simulink model "GridN1"  (R2021a)
settings: Solver=FixedStepAuto  StartTime=0  StopTime=0.2  FixedStep=0.2  RelTol=1e-3
libraries: spsDistributedParametersLineLib x45, spsThreePhaseSeriesRLCLoadLib x20, spsThreePhaseVIMeasurementLib x3, spsGroundLib x1, spsThreePhaseSourceLib x1, spsSeriesRLCBranchLib x1, spspowerguiLib x1
settings Model: Creator=miair  LastModifiedBy=Admin
settings SolverCC: AlgebraicLoopSolver=TrustRegion
settings DebuggingCC: SFMachineParentedDataDiag=warning  ArithmeticOperatorsInVariantConditions=warning
settings SFSimCC: SimUseLocalCustomCode=off  CustomCodeUndefinedFunction=UseInterfaceOnly
settings RTWCC: RTWUseLocalCustomCode=off
settings CodeAppCC: StateflowObjectComments=on
settings SimscapeCC: SimscapeNormalizeSystem=off

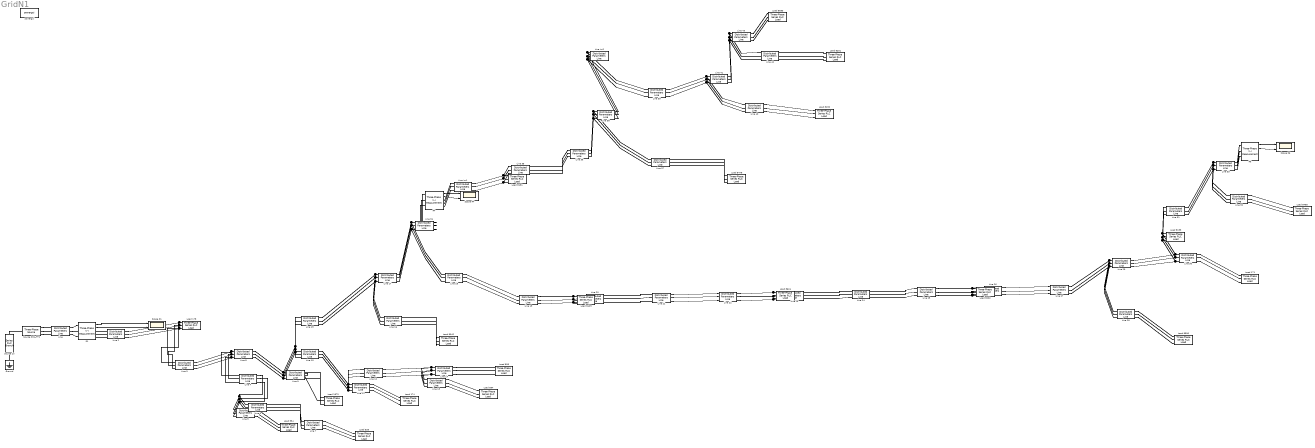
== system GridN1 ==
  Ground : spsGroundLib/Ground  LConnTagsString=a
  Line : spsDistributedParametersLineLib/Distributed Parameters Line  Phases=3  Length=0.01  Frequency=50  Resistance=[0.476003738225748 0.351747138225748 0.351747138225748;0.351747138225748 0.476003738225748 0.351747138225748;0.351747138225748 0.351747138225748 0.476003738225748]  Inductance=[0.000705954362986426 0.000459934243504405 0.000459934243504405;0.000459934243504405 0.000705954362986426 0.000459934243504405;0.000459934243504405 0.000459934243504405 0.000705954362986426]  Capacitance=[5.7561313269996e-07 -1.37543883484145e-07 -1.37543912800485e-07;-1.37543883484145e-07 5.75613027339387e-07 -1.37543875208088e-07;-1.37543912800485e-07 -1.37543875208088e-07 5.75613005057695e-07]  x1=[0.0222918353241703 9996.20639418684 9996.23586348623;314.159265358979 314.159265358979 314.159265358979;-2.28229478164881 -0.0972557313133246 -1.66804956884066]  x2=[0.0224219941863574 9996.18662579448 9996.21615012017;314.159265358979 314.159265358979 314.159265358979;-2.29395694441801 -0.0972566655221466 -1.6680505040101]  x3=[0.0226867751729249 523.332989705952 523.362905807898;314.159265358979 314.159265358979 314.159265358979;2.49195661502646 -0.0939976901170382 -1.66484033904786]  x4=[0.0226537478224017 553.014401101101 552.98741661978;314.159265358979 314.159265358979 314.159265358979;-0.676409249690145 -0.100380312178233 -1.67112828301793]  x5=2.2104317621921e-07  V1=[9.635 6853 6854;314.2 314.2 314.2;-1.242 -0.5939 -2.165]  V2=[9.699 6846 6847;314.2 314.2 314.2;-1.252 -0.5942 -2.166]  I1=[9.527 4746 4750;314.2 314.2 314.2;-2.657 2.284 0.7135]  I2=[9.488 5462 5466;314.2 314.2 314.2;0.457 -0.8227 -2.393]  nHarmo=1  Measurements=None  Decoupling=off  VsMag0=0  VrMag0=0  VsAngle0=0  VrAngle0=0  IsMag0=0  IrMag0=0  IsAngle0=0  IrAngle0=0
      settings: SourceProductBaseCode=PS
  Line 10 : spsDistributedParametersLineLib/Distributed Parameters Line  Phases=3  Length=0.16  Frequency=50  Resistance=[0.646656091154803 0.0486237908083191 0.0486712220507153;0.0486237908083191 0.646561225344642 0.0486237934466192;0.0486712220507153 0.0486237934466192 0.646656091154803]  Inductance=[0.00282448912315926 0.00133270803418135 0.00132951476746136;0.00133270803418135 0.00282479813276775 0.00133799988507366;0.00132951476746136 0.00133799988507366 0.00282448912315926]  Capacitance=[7.89543174552926e-09 -1.85986777702161e-09 -1.7901190036642e-09;-1.85986777702161e-09 7.82540023894543e-09 -1.8957321828871e-09;-1.7901190036642e-09 -1.8957321828871e-09 7.91264394645417e-09]  x1=[130.242577399402 9963.50829942501 9962.77347738552;314.159265358979 314.159265358979 314.159265358979;1.01854923332086 -0.181752113407925 -1.75268332597278]  x2=[130.243692976676 9963.37556751988 9962.64108071363;314.159265358979 314.159265358979 314.159265358979;1.01855097906876 -0.181754131846879 -1.75268530898728]  x3=[0.116077425207704 24.3976827501264 24.5901057255645;314.159265358979 314.159265358979 314.159265358979;0.991596864147124 -0.159547650801935 -1.73069418429352]  x4=[0.11174228141484 26.3164824795818 26.5095150382448;314.159265358979 314.159265358979 314.159265358979;1.04630376439903 -0.202523669719153 -1.7732666287694]  x5=7.66635634017784e-07  V1=[104 5068 5071;314.2 314.2 314.2;0.347 -0.922 -2.492]  V2=[104 5068 5071;314.2 314.2 314.2;0.347 -0.922 -2.492]  I1=[0.09471 11.28 11.38;314.2 314.2 314.2;0.3017 -0.8557 -2.427]  I2=[0.0873 14.56 14.67;314.2 314.2 314.2;0.3959 -0.9736 -2.543]  nHarmo=1  Measurements=None  Decoupling=off  VsMag0=0  VrMag0=0  VsAngle0=0  VrAngle0=0  IsMag0=0  IrMag0=0  IsAngle0=0  IrAngle0=0
      settings: SourceProductBaseCode=PS
  Line 11 : spsDistributedParametersLineLib/Distributed Parameters Line  Phases=3  Length=0.16  Frequency=50  Resistance=[0.646656091154803 0.0486237908083191 0.0486712220507153;0.0486237908083191 0.646561225344642 0.0486237934466192;0.0486712220507153 0.0486237934466192 0.646656091154803]  Inductance=[0.00282448912315926 0.00133270803418135 0.00132951476746136;0.00133270803418135 0.00282479813276775 0.00133799988507366;0.00132951476746136 0.00133799988507366 0.00282448912315926]  Capacitance=[7.89543174552926e-09 -1.85986777702161e-09 -1.7901190036642e-09;-1.85986777702161e-09 7.82540023894543e-09 -1.8957321828871e-09;-1.7901190036642e-09 -1.8957321828871e-09 7.91264394645417e-09]  x1=[130.243692976676 9963.37556751988 9962.64108071363;314.159265358979 314.159265358979 314.159265358979;1.01855097906876 -0.181754131846879 -1.75268530898728]  x2=[130.244363126695 9963.28020663524 9962.54594872537;314.159265358979 314.159265358979 314.159265358979;1.01855233432621 -0.181754623875762 -1.75268577248961]  x3=[0.115307169041535 24.7141260082062 24.9066741422531;314.159265358979 314.159265358979 314.159265358979;1.00266287682177 -0.163537863321983 -1.73461657859535]  x4=[0.112457939050156 25.9958508037535 26.1888200330395;314.159265358979 314.159265358979 314.159265358979;1.03459912527221 -0.19925926452526 -1.7700566377873]  x5=7.66635634017784e-07  V1=[104 5068 5071;314.2 314.2 314.2;0.347 -0.922 -2.492]  V2=[104 5068 5071;314.2 314.2 314.2;0.347 -0.922 -2.492]  I1=[0.09332 11.85 11.95;314.2 314.2 314.2;0.3203 -0.879 -2.45]  I2=[0.08855 13.96 14.07;314.2 314.2 314.2;0.375 -0.9588 -2.529]  nHarmo=1  Measurements=None  Decoupling=off  VsMag0=0  VrMag0=0  VsAngle0=0  VrAngle0=0  IsMag0=0  IrMag0=0  IsAngle0=0  IrAngle0=0
      settings: SourceProductBaseCode=PS
  Line 12 : spsDistributedParametersLineLib/Distributed Parameters Line  Phases=3  Length=0.18  Frequency=50  Resistance=[0.646656091154803 0.0486237908083191 0.0486712220507153;0.0486237908083191 0.646561225344642 0.0486237934466192;0.0486712220507153 0.0486237934466192 0.646656091154803]  Inductance=[0.00282448912315926 0.00133270803418135 0.00132951476746136;0.00133270803418135 0.00282479813276775 0.00133799988507366;0.00132951476746136 0.00133799988507366 0.00282448912315926]  Capacitance=[7.89543174552926e-09 -1.85986777702161e-09 -1.7901190036642e-09;-1.85986777702161e-09 7.82540023894543e-09 -1.8957321828871e-09;-1.7901190036642e-09 -1.8957321828871e-09 7.91264394645417e-09]  x1=[130.243692976676 9963.37556751988 9962.64108071363;314.159265358979 314.159265358979 314.159265358979;1.01852087335781 -0.181778048856944 -1.75270924876464]  x2=[130.244180802442 9963.33288399002 9962.59851563774;314.159265358979 314.159265358979 314.159265358979;1.01852135660549 -0.181779684234246 -1.75271087568807]  x3=[0.114617274330231 25.0319839397866 25.224671107872;314.159265358979 314.159265358979 314.159265358979;1.00745060338811 -0.177928318124719 -1.74892114944442]  x4=[0.113130219867099 25.6692741992299 25.8621448291562;314.159265358979 314.159265358979 314.159265358979;1.02946440993874 -0.185746412630351 -1.75661839923368]  x5=8.62465088270006e-07  V1=[104 5068 5071;314.2 314.2 314.2;0.347 -0.9221 -2.492]  V2=[104 5068 5071;314.2 314.2 314.2;0.347 -0.9221 -2.492]  I1=[0.09224 12.31 12.42;314.2 314.2 314.2;0.3278 -0.9025 -2.473]  I2=[0.08959 13.48 13.59;314.2 314.2 314.2;0.3665 -0.9401 -2.51]  nHarmo=1  Measurements=None  Decoupling=off  VsMag0=0  VrMag0=0  VsAngle0=0  VrAngle0=0  IsMag0=0  IrMag0=0  IsAngle0=0  IrAngle0=0
      settings: SourceProductBaseCode=PS
  Line 13 : spsDistributedParametersLineLib/Distributed Parameters Line  Phases=3  Length=0.52999  Frequency=50  Resistance=[0.646656091154803 0.0486237908083191 0.0486712220507153;0.0486237908083191 0.646561225344642 0.0486237934466192;0.0486712220507153 0.0486237934466192 0.646656091154803]  Inductance=[0.00282448912315926 0.00133270803418135 0.00132951476746136;0.00133270803418135 0.00282479813276775 0.00133799988507366;0.00132951476746136 0.00133799988507366 0.00282448912315926]  Capacitance=[7.89543174552926e-09 -1.85986777702161e-09 -1.7901190036642e-09;-1.85986777702161e-09 7.82540023894543e-09 -1.8957321828871e-09;-1.7901190036642e-09 -1.8957321828871e-09 7.91264394645417e-09]  x1=[130.244180802442 9963.33288399002 9962.59851563773;314.159265358979 314.159265358979 314.159265358979;1.01799452171676 -0.182198219951874 -1.75312980982207]  x2=[130.244900093266 9963.2358988461 9962.50174723082;314.159265358979 314.159265358979 314.159265358979;1.0179962481307 -0.182199789396365 -1.7531313496329]  x3=[0.114343695133595 25.1274088815328 25.31997383186;314.159265358979 314.159265358979 314.159265358979;1.01256874909253 -0.177815624881385 -1.74878775639587]  x4=[0.113355176518573 25.5534154820841 25.7461033654855;314.159265358979 314.159265358979 314.159265358979;1.02266801057171 -0.187137940104368 -1.75803079339372]  x5=2.53943262295678e-06  V1=[104 5068 5071;314.2 314.2 314.2;0.3465 -0.9225 -2.493]  V2=[104 5068 5071;314.2 314.2 314.2;0.3465 -0.9225 -2.493]  I1=[0.09195 12.42 12.53;314.2 314.2 314.2;0.3337 -0.9048 -2.475]  I2=[0.08984 13.36 13.47;314.2 314.2 314.2;0.3587 -0.9395 -2.51]  nHarmo=1  Measurements=None  Decoupling=off  VsMag0=0  VrMag0=0  VsAngle0=0  VrAngle0=0  IsMag0=0  IrMag0=0  IsAngle0=0  IrAngle0=0
      settings: SourceProductBaseCode=PS
  Line 14 : spsDistributedParametersLineLib/Distributed Parameters Line  Phases=3  Length=2.16  Frequency=50  Resistance=[0.646656091154803 0.0486237908083191 0.0486712220507153;0.0486237908083191 0.646561225344642 0.0486237934466192;0.0486712220507153 0.0486237934466192 0.646656091154803]  Inductance=[0.00282448912315926 0.00133270803418135 0.00132951476746136;0.00133270803418135 0.00282479813276775 0.00133799988507366;0.00132951476746136 0.00133799988507366 0.00282448912315926]  Capacitance=[7.89543174552926e-09 -1.85986777702161e-09 -1.7901190036642e-09;-1.85986777702161e-09 7.82540023894543e-09 -1.8957321828871e-09;-1.7901190036642e-09 -1.8957321828871e-09 7.91264394645417e-09]  x1=[130.244180802442 9963.33288399002 9962.59851563773;314.159265358979 314.159265358979 314.159265358979;1.01554089122167 -0.184147468230652 -1.75508091364718]  x2=[130.246188458181 9963.17178676299 9962.43787567194;314.159265358979 314.159265358979 314.159265358979;1.0155426828439 -0.184155057055003 -1.75508847407956]  x3=[0.114008072271456 25.1877940607526 25.3796823118794;314.159265358979 314.159265358979 314.159265358979;1.01012810506306 -0.184477664737353 -1.75543157329917]  x4=[0.11351032919889 25.3982164815801 25.5901584818446;314.159265358979 314.159265358979 314.159265358979;1.01771952031985 -0.186402015101581 -1.75731766205471]  x5=1.03495810592401e-05  V1=[104 5068 5071;314.2 314.2 314.2;0.344 -0.9244 -2.495]  V2=[104 5068 5071;314.2 314.2 314.2;0.344 -0.9245 -2.495]  I1=[0.09108 12.75 12.85;314.2 314.2 314.2;0.3377 -0.9226 -2.493]  I2=[0.09055 12.98 13.09;314.2 314.2 314.2;0.347 -0.9288 -2.499]  nHarmo=1  Measurements=None  Decoupling=off  VsMag0=0  VrMag0=0  VsAngle0=0  VrAngle0=0  IsMag0=0  IrMag0=0  IsAngle0=0  IrAngle0=0
      settings: SourceProductBaseCode=PS
  Line 15 : spsDistributedParametersLineLib/Distributed Parameters Line  Phases=3  Length=4.0599  Frequency=50  Resistance=[0.502970710632245 0.0486237908083191 0.0486712220507153;0.0486237908083191 0.502875844822084 0.0486237934466192;0.0486712220507153 0.0486237934466192 0.502970710632245]  Inductance=[0.00286900545038753 0.00133270803418135 0.00132951476746136;0.00133270803418135 0.00286931445999602 0.00133799988507366;0.00132951476746136 0.00133799988507366 0.00286900545038753]  Capacitance=[8.11484299003193e-09 -1.94249816214699e-09 -1.86930692621136e-09;-1.94249816214699e-09 8.0425699231653e-09 -1.98049571960044e-09;-1.86930692621136e-09 -1.98049571960044e-09 8.13337738722527e-09]  x1=[235.453514952772 9963.46848629237 9962.60262698438;314.159265358979 314.159265358979 314.159265358979;0.994594806145519 -0.180332661999128 -1.7512953556103]  x2=[235.289643988481 9940.78709251296 9940.03471226292;314.159265358979 314.159265358979 314.159265358979;0.994363051264843 -0.182485367956291 -1.75343150026667]  x3=[0.192916401807502 13.764259282743 13.9852677332489;314.159265358979 314.159265358979 314.159265358979;1.08672445935242 -0.13357416722545 -1.70691704016059]  x4=[0.220943474027241 36.7625568194615 36.9224157118885;314.159265358979 314.159265358979 314.159265358979;0.908177308687925 -0.202751798604677 -1.77302605148677]  x5=1.96600110340104e-05  V1=[157.3 5068 5071;314.2 314.2 314.2;0.3043 -0.9206 -2.491]  V2=[157.3 5040 5043;314.2 314.2 314.2;0.3032 -0.924 -2.494]  I1=[0.117 3.332 3.375;314.2 314.2 314.2;0.2152 0.2769 -1.319]  I2=[0.1593 24.64 24.76;314.2 314.2 314.2;0.3633 -1.051 -2.621]  nHarmo=1  Measurements=None  Decoupling=off  VsMag0=0  VrMag0=0  VsAngle0=0  VrAngle0=0  IsMag0=0  IrMag0=0  IsAngle0=0  IrAngle0=0
      settings: SourceProductBaseCode=PS
  Line 16 : spsDistributedParametersLineLib/Distributed Parameters Line  Phases=3  Length=0.01  Frequency=50  Resistance=[0.646656091154803 0.0486237908083191 0.0486712220507153;0.0486237908083191 0.646561225344642 0.0486237934466192;0.0486712220507153 0.0486237934466192 0.646656091154803]  Inductance=[0.00282448912315926 0.00133270803418135 0.00132951476746136;0.00133270803418135 0.00282479813276775 0.00133799988507366;0.00132951476746136 0.00133799988507366 0.00282448912315926]  Capacitance=[7.89543174552926e-09 -1.85986777702161e-09 -1.7901190036642e-09;-1.85986777702161e-09 7.82540023894543e-09 -1.8957321828871e-09;-1.7901190036642e-09 -1.8957321828871e-09 7.91264394645417e-09]  x1=[130.326330166885 9940.82738751096 9940.20612917528;314.159265358979 314.159265358979 314.159265358979;1.02002520165553 -0.183725424913734 -1.75463974696505]  x2=[130.326335050409 9940.82665087276 9940.20539375896;314.159265358979 314.159265358979 314.159265358979;1.02002522209908 -0.183725447358957 -1.75463976914281]  x3=[0.114182091967847 25.2037587974992 25.3964430297264;314.159265358979 314.159265358979 314.159265358979;1.01841585092938 -0.182271643264368 -1.75319795336006]  x4=[0.113714830492846 25.3923443415422 25.5850754232852;314.159265358979 314.159265358979 314.159265358979;1.02162610273495 -0.185180346028079 -1.75608285848536]  x5=4.79147271261115e-08  V1=[104.3 5040 5044;314.2 314.2 314.2;0.347 -0.9253 -2.495]  V2=[104.3 5040 5044;314.2 314.2 314.2;0.347 -0.9253 -2.495]  I1=[0.09135 12.75 12.86;314.2 314.2 314.2;0.3451 -0.9225 -2.493]  I2=[0.09103 12.9 13.01;314.2 314.2 314.2;0.3489 -0.928 -2.498]  nHarmo=1  Measurements=None  Decoupling=off  VsMag0=0  VrMag0=0  VsAngle0=0  VrAngle0=0  IsMag0=0  IrMag0=0  IsAngle0=0  IrAngle0=0
      settings: SourceProductBaseCode=PS
  Line 17 : spsDistributedParametersLineLib/Distributed Parameters Line  Phases=3  Length=0.35  Frequency=50  Resistance=[0.646656091154803 0.0486237908083191 0.0486712220507153;0.0486237908083191 0.646561225344642 0.0486237934466192;0.0486712220507153 0.0486237934466192 0.646656091154803]  Inductance=[0.00282448912315926 0.00133270803418135 0.00132951476746136;0.00133270803418135 0.00282479813276775 0.00133799988507366;0.00132951476746136 0.00133799988507366 0.00282448912315926]  Capacitance=[7.89543174552926e-09 -1.85986777702161e-09 -1.7901190036642e-09;-1.85986777702161e-09 7.82540023894543e-09 -1.8957321828871e-09;-1.7901190036642e-09 -1.8957321828871e-09 7.91264394645417e-09]  x1=[130.326330166885 9940.82738751096 9940.20612917528;314.159265358979 314.159265358979 314.159265358979;1.01951340456942 -0.184132014084834 -1.75504672318025]  x2=[130.326576288672 9938.31082064819 9937.70046419945;314.159265358979 314.159265358979 314.159265358979;1.01970088187677 -0.184306705852292 -1.75522007120294]  x3=[0.148957385141146 13.843926681644 14.0660841449284;314.159265358979 314.159265358979 314.159265358979;1.11614442248146 -0.132882540279348 -1.7060209099556]  x4=[0.0808905380770956 36.7514079439891 36.9126575942047;314.159265358979 314.159265358979 314.159265358979;0.840413226741481 -0.203838230701372 -1.77413120241162]  x5=1.6770154494139e-06  V1=[104.3 5040 5044;314.2 314.2 314.2;0.3465 -0.9257 -2.496]  V2=[104.3 5037 5041;314.2 314.2 314.2;0.3465 -0.9259 -2.496]  I1=[0.1199 3.328 3.373;314.2 314.2 314.2;0.1188 0.2711 -1.325]  I2=[0.0709 24.62 24.74;314.2 314.2 314.2;0.7375 -1.052 -2.622]  nHarmo=1  Measurements=None  Decoupling=off  VsMag0=0  VrMag0=0  VsAngle0=0  VrAngle0=0  IsMag0=0  IrMag0=0  IsAngle0=0  IrAngle0=0
      settings: SourceProductBaseCode=PS
  Line 18 : spsDistributedParametersLineLib/Distributed Parameters Line  Phases=3  Length=0.26  Frequency=50  Resistance=[0.646656091154803 0.0486237908083191 0.0486712220507153;0.0486237908083191 0.646561225344642 0.0486237934466192;0.0486712220507153 0.0486237934466192 0.646656091154803]  Inductance=[0.00282448912315926 0.00133270803418135 0.00132951476746136;0.00133270803418135 0.00282479813276775 0.00133799988507366;0.00132951476746136 0.00133799988507366 0.00282448912315926]  Capacitance=[7.89543174552926e-09 -1.85986777702161e-09 -1.7901190036642e-09;-1.85986777702161e-09 7.82540023894543e-09 -1.8957321828871e-09;-1.7901190036642e-09 -1.8957321828871e-09 7.91264394645417e-09]  x1=[130.326576288672 9938.31082064819 9937.70046419945;314.159265358979 314.159265358979 314.159265358979;1.01983635757603 -0.184199079307001 -1.7551123422048]  x2=[130.32916204716 9937.91496452812 9937.30324884027;314.159265358979 314.159265358979 314.159265358979;1.01988657290202 -0.184291336643042 -1.75520429655963]  x3=[0.128362374673362 20.9844255117936 21.1761964582734;314.159265358979 314.159265358979 314.159265358979;1.02313638417978 -0.299396844427883 -1.86945347333393]  x4=[0.099510978214805 29.8193505637966 30.0116107038491;314.159265358979 314.159265358979 314.159265358979;1.01518890877031 -0.103566007562585 -1.67486508115034]  x5=1.2457829052789e-06  V1=[104.3 5037 5041;314.2 314.2 314.2;0.3467 -0.9258 -2.496]  V2=[104.3 5037 5040;314.2 314.2 314.2;0.3467 -0.9259 -2.496]  I1=[0.1068 7.796 7.899;314.2 314.2 314.2;0.212 -0.9318 -2.502]  I2=[0.0779 17.83 17.94;314.2 314.2 314.2;0.5314 -0.9235 -2.494]  nHarmo=1  Measurements=None  Decoupling=off  VsMag0=0  VrMag0=0  VsAngle0=0  VrAngle0=0  IsMag0=0  IrMag0=0  IsAngle0=0  IrAngle0=0
      settings: SourceProductBaseCode=PS
  Line 19 : spsDistributedParametersLineLib/Distributed Parameters Line  Phases=3  Length=0.03  Frequency=50  Resistance=[0.476003738225748 0.351747138225748 0.351747138225748;0.351747138225748 0.476003738225748 0.351747138225748;0.351747138225748 0.351747138225748 0.476003738225748]  Inductance=[0.000705954362986426 0.000459934243504405 0.000459934243504405;0.000459934243504405 0.000705954362986426 0.000459934243504405;0.000459934243504405 0.000459934243504405 0.000705954362986426]  Capacitance=[5.7561313269996e-07 -1.37543883484145e-07 -1.37543912800485e-07;-1.37543883484145e-07 5.75613027339387e-07 -1.37543875208088e-07;-1.37543912800485e-07 -1.37543875208088e-07 5.75613005057695e-07]  x1=[1.4245093941287 9938.921477753 9939.26691274474;314.159265358979 314.159265358979 314.159265358979;1.82398634370718 -0.102457528041248 -1.67321690162597]  x2=[1.42447038511088 9938.91043185994 9939.25587007396;314.159265358979 314.159265358979 314.159265358979;1.82392224719724 -0.102459453209609 -1.67321882778548]  x3=[0.0175810099011775 530.600966790518 530.618889837519;314.159265358979 314.159265358979 314.159265358979;1.72300166696899 -0.106990520429841 -1.67775430675222]  x4=[0.0213020889565239 539.476384174009 539.495590731675;314.159265358979 314.159265358979 314.159265358979;1.90703711233556 -0.0981248397781654 -1.66887988222353]  x5=6.63129528657629e-07  V1=[39.29 5037 5041;314.2 314.2 314.2;0.4733 -0.844 -2.414]  V2=[39.29 5037 5041;314.2 314.2 314.2;0.4733 -0.844 -2.414]  I1=[0.5337 266.1 266.4;314.2 314.2 314.2;0.4559 -0.8442 -2.414]  I2=[0.5344 276.2 276.4;314.2 314.2 314.2;0.4906 -0.844 -2.414]  nHarmo=1  Measurements=None  Decoupling=off  VsMag0=0  VrMag0=0  VsAngle0=0  VrAngle0=0  IsMag0=0  IrMag0=0  IsAngle0=0  IrAngle0=0
      settings: SourceProductBaseCode=PS
  Line 2 : spsDistributedParametersLineLib/Distributed Parameters Line  Phases=3  Length=0.61194  Frequency=50  Resistance=[0.502970710632245 0.0486237908083191 0.0486712220507153;0.0486237908083191 0.502875844822084 0.0486237934466192;0.0486712220507153 0.0486237934466192 0.502970710632245]  Inductance=[0.00286900545038753 0.00133270803418135 0.00132951476746136;0.00133270803418135 0.00286931445999602 0.00133799988507366;0.00132951476746136 0.00133799988507366 0.00286900545038753]  Capacitance=[8.11484299003193e-09 -1.94249816214699e-09 -1.86930692621136e-09;-1.94249816214699e-09 8.0425699231653e-09 -1.98049571960044e-09;-1.86930692621136e-09 -1.98049571960044e-09 8.13337738722527e-09]  x1=[235.621244120723 9995.10614951882 9994.09853412887;314.159265358979 314.159265358979 314.159265358979;1.00026286084811 -0.173384388263363 -1.7443628648723]  x2=[235.598383234402 9990.4663688478 9989.47907733026;314.159265358979 314.159265358979 314.159265358979;1.00019786045036 -0.17377601649056 -1.74475153846886]  x3=[0.187652092361818 10.7368768875938 10.9525674806308;314.159265358979 314.159265358979 314.159265358979;1.07865741182198 -0.0117777434078454 -1.58843679844733]  x4=[0.226610082018719 40.3022239606716 40.4637821834707;314.159265358979 314.159265358979 314.159265358979;0.934456544180452 -0.216987397055439 -1.78713462567906]  x5=2.96331120277651e-06  V1=[159.9 6845 6846;314.2 314.2 314.2;0.4431 -0.6704 -2.242]  V2=[157.3 5087 5090;314.2 314.2 314.2;0.3101 -0.9143 -2.485]  I1=[17.14 5085 5089;314.2 314.2 314.2;-2.556 2.225 0.6553]  I2=[17.41 5115 5119;314.2 314.2 314.2;0.5825 -0.9156 -2.485]  nHarmo=1  Measurements=None  Decoupling=off  VsMag0=0  VrMag0=0  VsAngle0=0  VrAngle0=0  IsMag0=0  IrMag0=0  IsAngle0=0  IrAngle0=0
      settings: SourceProductBaseCode=PS
  Line 20 : spsDistributedParametersLineLib/Distributed Parameters Line  Phases=3  Length=0.06  Frequency=50  Resistance=[0.476003738225748 0.351747138225748 0.351747138225748;0.351747138225748 0.476003738225748 0.351747138225748;0.351747138225748 0.351747138225748 0.476003738225748]  Inductance=[0.000705954362986426 0.000459934243504405 0.000459934243504405;0.000459934243504405 0.000705954362986426 0.000459934243504405;0.000459934243504405 0.000459934243504405 0.000705954362986426]  Capacitance=[5.7561313269996e-07 -1.37543883484145e-07 -1.37543912800485e-07;-1.37543883484145e-07 5.75613027339387e-07 -1.37543875208088e-07;-1.37543912800485e-07 -1.37543875208088e-07 5.75613005057695e-07]  x1=[1.42447038511088 9938.91043185994 9939.25587007396;314.159265358979 314.159265358979 314.159265358979;1.82371391891168 -0.102584291845602 -1.67334366641182]  x2=[1.4243921983318 9938.89251201755 9939.23795682133;314.159265358979 314.159265358979 314.159265358979;1.82358601554388 -0.102588056799812 -1.67334743334833]  x3=[0.0175736449417827 530.975678012254 530.993615230172;314.159265358979 314.159265358979 314.159265358979;1.72293473985058 -0.107494540348251 -1.67825832448805]  x4=[0.0212927276916265 538.94061145443 538.959800320809;314.159265358979 314.159265358979 314.159265358979;1.90634883674491 -0.0979982060947546 -1.66875324680576]  x5=1.32625905731526e-06  V1=[39.29 5037 5041;314.2 314.2 314.2;0.4731 -0.8442 -2.414]  V2=[39.29 5037 5041;314.2 314.2 314.2;0.4731 -0.8442 -2.414]  I1=[0.5336 266.8 267;314.2 314.2 314.2;0.4559 -0.8455 -2.416]  I2=[0.5343 275.4 275.6;314.2 314.2 314.2;0.4899 -0.8431 -2.413]  nHarmo=1  Measurements=None  Decoupling=off  VsMag0=0  VrMag0=0  VsAngle0=0  VrAngle0=0  IsMag0=0  IrMag0=0  IsAngle0=0  IrAngle0=0
      settings: SourceProductBaseCode=PS
  Line 21 : spsDistributedParametersLineLib/Distributed Parameters Line  Phases=3  Length=0.2  Frequency=50  Resistance=[0.646656091154803 0.0486237908083191 0.0486712220507153;0.0486237908083191 0.646561225344642 0.0486237934466192;0.0486712220507153 0.0486237934466192 0.646656091154803]  Inductance=[0.00282448912315926 0.00133270803418135 0.00132951476746136;0.00133270803418135 0.00282479813276775 0.00133799988507366;0.00132951476746136 0.00133799988507366 0.00282448912315926]  Capacitance=[7.89543174552926e-09 -1.85986777702161e-09 -1.7901190036642e-09;-1.85986777702161e-09 7.82540023894543e-09 -1.8957321828871e-09;-1.7901190036642e-09 -1.8957321828871e-09 7.91264394645417e-09]  x1=[130.3288950013 9937.88599990961 9937.27430099486;314.159265358979 314.159265358979 314.159265358979;1.01996916243804 -0.184225275841895 -1.75513817028224]  x2=[130.33048890442 9937.64171575033 9937.02891559282;314.159265358979 314.159265358979 314.159265358979;1.02000525610896 -0.184292692646946 -1.75520537945401]  x3=[0.127146014419732 21.4436534566221 21.6354893278325;314.159265358979 314.159265358979 314.159265358979;1.02820850828029 -0.29982856907374 -1.8698903160141]  x4=[0.100745489126736 29.3726424076949 29.5647865107489;314.159265358979 314.159265358979 314.159265358979;1.0092709177691 -0.100181363095939 -1.67151361214128]  x5=9.5829454252223e-07  V1=[104.3 5037 5040;314.2 314.2 314.2;0.3468 -0.9259 -2.496]  V2=[104.3 5036 5039;314.2 314.2 314.2;0.3468 -0.9259 -2.496]  I1=[0.1048 8.53 8.633;314.2 314.2 314.2;0.2269 -0.9605 -2.531]  I2=[0.07936 17.11 17.22;314.2 314.2 314.2;0.5051 -0.9088 -2.479]  nHarmo=1  Measurements=None  Decoupling=off  VsMag0=0  VrMag0=0  VsAngle0=0  VrAngle0=0  IsMag0=0  IrMag0=0  IsAngle0=0  IrAngle0=0
      settings: SourceProductBaseCode=PS
  Line 22 : spsDistributedParametersLineLib/Distributed Parameters Line  Phases=3  Length=0.05  Frequency=50  Resistance=[0.476003738225748 0.351747138225748 0.351747138225748;0.351747138225748 0.476003738225748 0.351747138225748;0.351747138225748 0.351747138225748 0.476003738225748]  Inductance=[0.000705954362986426 0.000459934243504405 0.000459934243504405;0.000459934243504405 0.000705954362986426 0.000459934243504405;0.000459934243504405 0.000459934243504405 0.000705954362986426]  Capacitance=[5.7561313269996e-07 -1.37543883484145e-07 -1.37543912800485e-07;-1.37543883484145e-07 5.75613027339387e-07 -1.37543875208088e-07;-1.37543912800485e-07 -1.37543875208088e-07 5.75613005057695e-07]  x1=[1.43742667692932 9938.64804771292 9938.99267639042;314.159265358979 314.159265358979 314.159265358979;1.82768376352005 -0.102613870488766 -1.67337302407057]  x2=[1.4373623164658 9938.63261999789 9938.9772540149;314.159265358979 314.159265358979 314.159265358979;1.8275806492845 -0.102616927803817 -1.67337608300181]  x3=[0.0177798667718985 530.987767813953 531.005671687073;314.159265358979 314.159265358979 314.159265358979;1.73073751005659 -0.107261738044963 -1.678025204756]  x4=[0.0214335988134183 538.952903514138 538.972038747062;314.159265358979 314.159265358979 314.159265358979;1.90765271050702 -0.0982442726964839 -1.66899918648451]  x5=1.10521588109605e-06  V1=[39.31 5036 5041;314.2 314.2 314.2;0.4733 -0.8442 -2.414]  V2=[39.31 5036 5041;314.2 314.2 314.2;0.4733 -0.8442 -2.414]  I1=[0.5338 266.8 267;314.2 314.2 314.2;0.4566 -0.8453 -2.416]  I2=[0.5345 275.4 275.6;314.2 314.2 314.2;0.4897 -0.8434 -2.414]  nHarmo=1  Measurements=None  Decoupling=off  VsMag0=0  VrMag0=0  VsAngle0=0  VrAngle0=0  IsMag0=0  IrMag0=0  IsAngle0=0  IrAngle0=0
      settings: SourceProductBaseCode=PS
  Line 23 : spsDistributedParametersLineLib/Distributed Parameters Line  Phases=3  Length=0.05  Frequency=50  Resistance=[0.476003738225748 0.351747138225748 0.351747138225748;0.351747138225748 0.476003738225748 0.351747138225748;0.351747138225748 0.351747138225748 0.476003738225748]  Inductance=[0.000705954362986426 0.000459934243504405 0.000459934243504405;0.000459934243504405 0.000705954362986426 0.000459934243504405;0.000459934243504405 0.000459934243504405 0.000705954362986426]  Capacitance=[5.7561313269996e-07 -1.37543883484145e-07 -1.37543912800485e-07;-1.37543883484145e-07 5.75613027339387e-07 -1.37543875208088e-07;-1.37543912800485e-07 -1.37543875208088e-07 5.75613005057695e-07]  x1=[1.4373623164658 9938.63261999789 9938.9772540149;314.159265358979 314.159265358979 314.159265358979;1.8275806492845 -0.102616927803817 -1.67337608300181]  x2=[1.43729779741554 9938.62081848283 9938.96545796523;314.159265358979 314.159265358979 314.159265358979;1.82747780372761 -0.102619837132001 -1.67337899394621]  x3=[0.0177785243799084 531.514289675707 531.532212515172;314.159265358979 314.159265358979 314.159265358979;1.73099929049252 -0.10743150921611 -1.67819497347757]  x4=[0.0214320357497241 538.425752294805 538.444869950834;314.159265358979 314.159265358979 314.159265358979;1.90724737882514 -0.0980737857836584 -1.66882869713321]  x5=1.10521588109605e-06  V1=[39.31 5036 5041;314.2 314.2 314.2;0.4733 -0.8442 -2.414]  V2=[39.31 5036 5041;314.2 314.2 314.2;0.4733 -0.8442 -2.414]  I1=[0.5338 267.5 267.8;314.2 314.2 314.2;0.4569 -0.8464 -2.417]  I2=[0.5345 274.6 274.9;314.2 314.2 314.2;0.4894 -0.8423 -2.412]  nHarmo=1  Measurements=None  Decoupling=off  VsMag0=0  VrMag0=0  VsAngle0=0  VrAngle0=0  IsMag0=0  IrMag0=0  IsAngle0=0  IrAngle0=0
      settings: SourceProductBaseCode=PS
  Line 24 : spsDistributedParametersLineLib/Distributed Parameters Line  Phases=3  Length=0.07  Frequency=50  Resistance=[0.646656091154803 0.0486237908083191 0.0486712220507153;0.0486237908083191 0.646561225344642 0.0486237934466192;0.0486712220507153 0.0486237934466192 0.646656091154803]  Inductance=[0.00282448912315926 0.00133270803418135 0.00132951476746136;0.00133270803418135 0.00282479813276775 0.00133799988507366;0.00132951476746136 0.00133799988507366 0.00282448912315926]  Capacitance=[7.89543174552926e-09 -1.85986777702161e-09 -1.7901190036642e-09;-1.85986777702161e-09 7.82540023894543e-09 -1.8957321828871e-09;-1.7901190036642e-09 -1.8957321828871e-09 7.91264394645417e-09]  x1=[130.330253366141 9937.61448730251 9937.00170510559;314.159265358979 314.159265358979 314.159265358979;1.0201927594141 -0.184143198840608 -1.75505574073195]  x2=[130.330683020795 9937.55025889592 9936.93708929831;314.159265358979 314.159265358979 314.159265358979;1.0202041668404 -0.184164948700032 -1.75507742846588]  x3=[0.125655201584127 21.9672135725545 22.1592091151028;314.159265358979 314.159265358979 314.159265358979;1.03192200208027 -0.295801486307576 -1.86590749201526]  x4=[0.102261420626483 28.8494546211149 29.04156551678;314.159265358979 314.159265358979 314.159265358979;1.00567540056309 -0.0992889931624274 -1.6706394067094]  x5=3.3540308988278e-07  V1=[104.3 5036 5039;314.2 314.2 314.2;0.347 -0.9258 -2.496]  V2=[104.3 5036 5039;314.2 314.2 314.2;0.347 -0.9258 -2.496]  I1=[0.1028 9.27 9.374;314.2 314.2 314.2;0.2424 -0.9834 -2.553]  I2=[0.08089 16.38 16.49;314.2 314.2 314.2;0.48 -0.8933 -2.464]  nHarmo=1  Measurements=None  Decoupling=off  VsMag0=0  VrMag0=0  VsAngle0=0  VrAngle0=0  IsMag0=0  IrMag0=0  IsAngle0=0  IrAngle0=0
      settings: SourceProductBaseCode=PS
  Line 25 : spsDistributedParametersLineLib/Distributed Parameters Line  Phases=3  Length=0.28  Frequency=50  Resistance=[0.476003738225748 0.351747138225748 0.351747138225748;0.351747138225748 0.476003738225748 0.351747138225748;0.351747138225748 0.351747138225748 0.476003738225748]  Inductance=[0.000705954362986426 0.000459934243504405 0.000459934243504405;0.000459934243504405 0.000705954362986426 0.000459934243504405;0.000459934243504405 0.000459934243504405 0.000705954362986426]  Capacitance=[5.7561313269996e-07 -1.37543883484145e-07 -1.37543912800485e-07;-1.37543883484145e-07 5.75613027339387e-07 -1.37543875208088e-07;-1.37543912800485e-07 -1.37543875208088e-07 5.75613005057695e-07]  x1=[1.44129723458618 9938.55653733702 9938.90087573775;314.159265358979 314.159265358979 314.159265358979;1.82728932314649 -0.103598686586373 -1.67435777574891]  x2=[1.44093492721902 9938.48245689733 9938.82682536803;314.159265358979 314.159265358979 314.159265358979;1.8267242754704 -0.103613685634719 -1.6743727837784]  x3=[0.0177909221646994 530.89542961591 530.913318724292;314.159265358979 314.159265358979 314.159265358979;1.7320984568824 -0.108201832285522 -1.67896519852232]  x4=[0.0214071248068408 537.796141081181 537.815215966937;314.159265358979 314.159265358979 314.159265358979;1.9040650343063 -0.100227736406211 -1.67098261923912]  x5=6.18920893413787e-06  V1=[39.31 5036 5040;314.2 314.2 314.2;0.4718 -0.8452 -2.415]  V2=[39.31 5036 5040;314.2 314.2 314.2;0.4717 -0.8452 -2.415]  I1=[0.5324 267.2 267.4;314.2 314.2 314.2;0.4557 -0.8472 -2.417]  I2=[0.5331 274.3 274.6;314.2 314.2 314.2;0.4858 -0.8444 -2.415]  nHarmo=1  Measurements=None  Decoupling=off  VsMag0=0  VrMag0=0  VsAngle0=0  VrAngle0=0  IsMag0=0  IrMag0=0  IsAngle0=0  IrAngle0=0
      settings: SourceProductBaseCode=PS
  Line 26 : spsDistributedParametersLineLib/Distributed Parameters Line  Phases=3  Length=0.28  Frequency=50  Resistance=[0.476003738225748 0.351747138225748 0.351747138225748;0.351747138225748 0.476003738225748 0.351747138225748;0.351747138225748 0.351747138225748 0.476003738225748]  Inductance=[0.000705954362986426 0.000459934243504405 0.000459934243504405;0.000459934243504405 0.000705954362986426 0.000459934243504405;0.000459934243504405 0.000459934243504405 0.000705954362986426]  Capacitance=[5.7561313269996e-07 -1.37543883484145e-07 -1.37543912800485e-07;-1.37543883484145e-07 5.75613027339387e-07 -1.37543875208088e-07;-1.37543912800485e-07 -1.37543875208088e-07 5.75613005057695e-07]  x1=[1.44093492721902 9938.48245689733 9938.82682536803;314.159265358979 314.159265358979 314.159265358979;1.8267242754704 -0.103613685634719 -1.6743727837784]  x2=[1.44056762027621 9938.4341675694 9938.77856700824;314.159265358979 314.159265358979 314.159265358979;1.8261676694835 -0.103625539556922 -1.67438464668211]  x3=[0.0177834784353123 531.826655427082 531.844577248;314.159265358979 314.159265358979 314.159265358979;1.73358165613611 -0.107616396884259 -1.67837976428211]  x4=[0.0213984497798403 536.856011577801 536.87505428311;314.159265358979 314.159265358979 314.159265358979;1.9018067401518 -0.100820516922772 -1.67157540065818]  x5=6.18920893413787e-06  V1=[39.31 5036 5040;314.2 314.2 314.2;0.4717 -0.8452 -2.415]  V2=[39.31 5036 5040;314.2 314.2 314.2;0.4716 -0.8452 -2.415]  I1=[0.5324 268.4 268.6;314.2 314.2 314.2;0.4576 -0.8481 -2.418]  I2=[0.5331 273.1 273.4;314.2 314.2 314.2;0.4838 -0.8435 -2.414]  nHarmo=1  Measurements=None  Decoupling=off  VsMag0=0  VrMag0=0  VsAngle0=0  VrAngle0=0  IsMag0=0  IrMag0=0  IsAngle0=0  IrAngle0=0
      settings: SourceProductBaseCode=PS
  Line 27 : spsDistributedParametersLineLib/Distributed Parameters Line  Phases=3  Length=1.3599  Frequency=50  Resistance=[0.646656091154803 0.0486237908083191 0.0486712220507153;0.0486237908083191 0.646561225344642 0.0486237934466192;0.0486712220507153 0.0486237934466192 0.646656091154803]  Inductance=[0.00282448912315926 0.00133270803418135 0.00132951476746136;0.00133270803418135 0.00282479813276775 0.00133799988507366;0.00132951476746136 0.00133799988507366 0.00282448912315926]  Capacitance=[7.89543174552926e-09 -1.85986777702161e-09 -1.7901190036642e-09;-1.85986777702161e-09 7.82540023894543e-09 -1.8957321828871e-09;-1.7901190036642e-09 -1.8957321828871e-09 7.91264394645417e-09]  x1=[130.329728376385 9937.42789052548 9936.8148189084;314.159265358979 314.159265358979 314.159265358979;1.01822333703732 -0.185734329882512 -1.7566482950887]  x2=[130.338496259868 9936.32927121171 9935.71215355795;314.159265358979 314.159265358979 314.159265358979;1.01836969953116 -0.186018035051001 -1.75693116269203]  x3=[0.122105069941512 22.7827439363444 22.9746342104793;314.159265358979 314.159265358979 314.159265358979;1.01567753441308 -0.251864079284913 -1.82236470241038]  x4=[0.105655883762807 27.8033766478159 27.995277135231;314.159265358979 314.159265358979 314.159265358979;1.01911637520771 -0.133296733389247 -1.70446962376381]  x5=6.5159237418799e-06  V1=[104.3 5036 5039;314.2 314.2 314.2;0.345 -0.9274 -2.498]  V2=[104.4 5034 5037;314.2 314.2 314.2;0.3451 -0.9278 -2.498]  I1=[0.09898 10.42 10.52;314.2 314.2 314.2;0.2676 -0.9722 -2.542]  I2=[0.08401 15.19 15.3;314.2 314.2 314.2;0.4341 -0.8984 -2.469]  nHarmo=1  Measurements=None  Decoupling=off  VsMag0=0  VrMag0=0  VsAngle0=0  VrAngle0=0  IsMag0=0  IrMag0=0  IsAngle0=0  IrAngle0=0
      settings: SourceProductBaseCode=PS
  Line 28 : spsDistributedParametersLineLib/Distributed Parameters Line  Phases=3  Length=1.36  Frequency=50  Resistance=[0.646656091154803 0.0486237908083191 0.0486712220507153;0.0486237908083191 0.646561225344642 0.0486237934466192;0.0486712220507153 0.0486237934466192 0.646656091154803]  Inductance=[0.00282448912315926 0.00133270803418135 0.00132951476746136;0.00133270803418135 0.00282479813276775 0.00133799988507366;0.00132951476746136 0.00133799988507366 0.00282448912315926]  Capacitance=[7.89543174552926e-09 -1.85986777702161e-09 -1.7901190036642e-09;-1.85986777702161e-09 7.82540023894543e-09 -1.8957321828871e-09;-1.7901190036642e-09 -1.8957321828871e-09 7.91264394645417e-09]  x1=[130.338496259868 9936.32927121171 9935.71215355795;314.159265358979 314.159265358979 314.159265358979;1.01836954900261 -0.186018154636051 -1.75693128239092]  x2=[130.340101820962 9936.14779190958 9935.53111055935;314.159265358979 314.159265358979 314.159265358979;1.01837234852511 -0.1860225895451 -1.75693566845385]  x3=[0.114266435345695 25.083588878017 25.2755793368666;314.159265358979 314.159265358979 314.159265358979;1.01278704597775 -0.183852639034294 -1.75479750038726]  x4=[0.113505620900049 25.4115036632594 25.6035883430237;314.159265358979 314.159265358979 314.159265358979;1.02193777726997 -0.189776831341686 -1.760660406496]  x5=6.51640288915116e-06  V1=[104.4 5034 5037;314.2 314.2 314.2;0.3451 -0.9278 -2.498]  V2=[104.4 5034 5037;314.2 314.2 314.2;0.3451 -0.9278 -2.498]  I1=[0.09185 12.5 12.61;314.2 314.2 314.2;0.3356 -0.9181 -2.488]  I2=[0.09054 13.08 13.19;314.2 314.2 314.2;0.3527 -0.9386 -2.509]  nHarmo=1  Measurements=None  Decoupling=off  VsMag0=0  VrMag0=0  VsAngle0=0  VrAngle0=0  IsMag0=0  IrMag0=0  IsAngle0=0  IrAngle0=0
      settings: SourceProductBaseCode=PS
  Line 29 : spsDistributedParametersLineLib/Distributed Parameters Line  Phases=3  Length=0.17  Frequency=50  Resistance=[0.646656091154803 0.0486237908083191 0.0486712220507153;0.0486237908083191 0.646561225344642 0.0486237934466192;0.0486712220507153 0.0486237934466192 0.646656091154803]  Inductance=[0.00282448912315926 0.00133270803418135 0.00132951476746136;0.00133270803418135 0.00282479813276775 0.00133799988507366;0.00132951476746136 0.00133799988507366 0.00282448912315926]  Capacitance=[7.89543174552926e-09 -1.85986777702161e-09 -1.7901190036642e-09;-1.85986777702161e-09 7.82540023894543e-09 -1.8957321828871e-09;-1.7901190036642e-09 -1.8957321828871e-09 7.91264394645417e-09]  x1=[130.338496259868 9936.32927121171 9935.71215355795;314.159265358979 314.159265358979 314.159265358979;1.02016083880399 -0.184595092537201 -1.75550686563772]  x2=[130.339319282556 9936.21118379325 9935.59349904349;314.159265358979 314.159265358979 314.159265358979;1.02017902421298 -0.184629561336896 -1.75554123206193]  x3=[0.121802034104778 22.9772614099099 23.1696223349729;314.159265358979 314.159265358979 314.159265358979;1.02475203194087 -0.250832701105956 -1.82130088184292]  x4=[0.106101734358237 27.6782344120133 27.8705802010828;314.159265358979 314.159265358979 314.159265358979;1.01463495372603 -0.129837552175695 -1.70104033425866]  x5=8.14550361143895e-07  V1=[104.4 5034 5037;314.2 314.2 314.2;0.3469 -0.9264 -2.497]  V2=[104.4 5034 5037;314.2 314.2 314.2;0.3469 -0.9264 -2.497]  I1=[0.09832 10.72 10.83;314.2 314.2 314.2;0.2798 -0.9793 -2.549]  I2=[0.08464 14.92 15.03;314.2 314.2 314.2;0.4246 -0.8885 -2.459]  nHarmo=1  Measurements=None  Decoupling=off  VsMag0=0  VrMag0=0  VsAngle0=0  VrAngle0=0  IsMag0=0  IrMag0=0  IsAngle0=0  IrAngle0=0
      settings: SourceProductBaseCode=PS
  Line 3 : spsDistributedParametersLineLib/Distributed Parameters Line  Phases=3  Length=2.5878  Frequency=50  Resistance=[0.502970710632245 0.0486237908083191 0.0486712220507153;0.0486237908083191 0.502875844822084 0.0486237934466192;0.0486712220507153 0.0486237934466192 0.502970710632245]  Inductance=[0.00286900545038753 0.00133270803418135 0.00132951476746136;0.00133270803418135 0.00286931445999602 0.00133799988507366;0.00132951476746136 0.00133799988507366 0.00286900545038753]  Capacitance=[8.11484299003193e-09 -1.94249816214699e-09 -1.86930692621136e-09;-1.94249816214699e-09 8.0425699231653e-09 -1.98049571960044e-09;-1.86930692621136e-09 -1.98049571960044e-09 8.13337738722527e-09]  x1=[235.598383234402 9990.46636884779 9989.47907733026;314.159265358979 314.159265358979 314.159265358979;0.997191960905206 -0.176210407895843 -1.74718866951073]  x2=[235.499919862763 9971.07620664183 9970.17375086974;314.159265358979 314.159265358979 314.159265358979;0.996925146531869 -0.177855842884864 -1.74882161850263]  x3=[0.187754497029636 10.8325516761511 11.0482274955793;314.159265358979 314.159265358979 314.159265358979;1.07645890900216 -0.0226877727987938 -1.59910610362351]  x4=[0.226150622574205 40.0470654635873 40.2076661353264;314.159265358979 314.159265358979 314.159265358979;0.927558268141239 -0.220650358783432 -1.79081026181661]  x5=1.25313866237622e-05  V1=[157.3 5087 5090;314.2 314.2 314.2;0.3098 -0.9146 -2.485]  V2=[157.3 5078 5081;314.2 314.2 314.2;0.3094 -0.9156 -2.486]  I1=[0.1093 6.229 6.183;314.2 314.2 314.2;0.1996 1.242 -0.3409]  I2=[0.1676 29.77 29.89;314.2 314.2 314.2;0.3802 -1.091 -2.661]  nHarmo=1  Measurements=None  Decoupling=off  VsMag0=0  VrMag0=0  VsAngle0=0  VrAngle0=0  IsMag0=0  IrMag0=0  IsAngle0=0  IrAngle0=0
      settings: SourceProductBaseCode=PS
  Line 30 : spsDistributedParametersLineLib/Distributed Parameters Line  Phases=3  Length=1.32  Frequency=50  Resistance=[0.476003738225748 0.351747138225748 0.351747138225748;0.351747138225748 0.476003738225748 0.351747138225748;0.351747138225748 0.351747138225748 0.476003738225748]  Inductance=[0.000705954362986426 0.000459934243504405 0.000459934243504405;0.000459934243504405 0.000705954362986426 0.000459934243504405;0.000459934243504405 0.000459934243504405 0.000705954362986426]  Capacitance=[5.7561313269996e-07 -1.37543883484145e-07 -1.37543912800485e-07;-1.37543883484145e-07 5.75613027339387e-07 -1.37543875208088e-07;-1.37543912800485e-07 -1.37543875208088e-07 5.75613005057695e-07]  x1=[1.50379048684022 9937.21663670315 9937.55768878126;314.159265358979 314.159265358979 314.159265358979;1.83520307349907 -0.108271494958229 -1.67902959751446]  x2=[1.50385367637334 9937.27099515115 9937.6120490717;314.159265358979 314.159265358979 314.159265358979;1.83510606328783 -0.108295960837469 -1.67905406338995]  x3=[0.0201243032149866 531.074694626638 531.092880655042;314.159265358979 314.159265358979 314.159265358979;1.82598830604994 -0.113308456258091 -1.6840665583512]  x4=[0.020124284875677 531.918868616967 531.937083618422;314.159265358979 314.159265358979 314.159265358979;1.83510588000721 -0.1087676324025 -1.67952573499144]  x5=2.91776992609357e-05  V1=[39.37 5034 5038;314.2 314.2 314.2;0.4652 -0.85 -2.42]  V2=[39.37 5034 5038;314.2 314.2 314.2;0.4651 -0.85 -2.42]  I1=[0.5269 268.8 269;314.2 314.2 314.2;0.456 -0.8547 -2.425]  I2=[0.5269 269.7 269.9;314.2 314.2 314.2;0.4651 -0.8509 -2.421]  nHarmo=1  Measurements=None  Decoupling=off  VsMag0=0  VrMag0=0  VsAngle0=0  VrAngle0=0  IsMag0=0  IrMag0=0  IsAngle0=0  IrAngle0=0
      settings: SourceProductBaseCode=PS
  Line 31 : spsDistributedParametersLineLib/Distributed Parameters Line  Phases=3  Length=1.33  Frequency=50  Resistance=[0.646656091154803 0.0486237908083191 0.0486712220507153;0.0486237908083191 0.646561225344642 0.0486237934466192;0.0486712220507153 0.0486237934466192 0.646656091154803]  Inductance=[0.00282448912315926 0.00133270803418135 0.00132951476746136;0.00133270803418135 0.00282479813276775 0.00133799988507366;0.00132951476746136 0.00133799988507366 0.00282448912315926]  Capacitance=[7.89543174552926e-09 -1.85986777702161e-09 -1.7901190036642e-09;-1.85986777702161e-09 7.82540023894543e-09 -1.8957321828871e-09;-1.7901190036642e-09 -1.8957321828871e-09 7.91264394645417e-09]  x1=[130.339319282556 9936.21118379325 9935.59349904349;314.159265358979 314.159265358979 314.159265358979;1.01843289297802 -0.186016747920649 -1.75692973914909]  x2=[130.34485518947 9935.82252110572 9935.20612774522;314.159265358979 314.159265358979 314.159265358979;1.01843401913806 -0.186034740422742 -1.75694768905571]  x3=[0.114838955898379 24.8373909596553 25.0293061590383;314.159265358979 314.159265358979 314.159265358979;0.999898131821761 -0.18286370122636 -1.75386736418759]  x4=[0.112974507215708 25.6584639184276 25.8506292818783;314.159265358979 314.159265358979 314.159265358979;1.03525571867904 -0.190652425656919 -1.76147998391516]  x5=6.37265870777283e-06  V1=[104.4 5034 5037;314.2 314.2 314.2;0.3452 -0.9278 -2.498]  V2=[104.4 5033 5037;314.2 314.2 314.2;0.3452 -0.9278 -2.498]  I1=[0.09226 12.33 12.43;314.2 314.2 314.2;0.3242 -0.917 -2.487]  I2=[0.09017 13.26 13.36;314.2 314.2 314.2;0.3646 -0.9393 -2.509]  nHarmo=1  Measurements=None  Decoupling=off  VsMag0=0  VrMag0=0  VsAngle0=0  VrAngle0=0  IsMag0=0  IrMag0=0  IsAngle0=0  IrAngle0=0
      settings: SourceProductBaseCode=PS
  Line 32 : spsDistributedParametersLineLib/Distributed Parameters Line  Phases=3  Length=0.18  Frequency=50  Resistance=[0.646656091154803 0.0486237908083191 0.0486712220507153;0.0486237908083191 0.646561225344642 0.0486237934466192;0.0486712220507153 0.0486237934466192 0.646656091154803]  Inductance=[0.00282448912315926 0.00133270803418135 0.00132951476746136;0.00133270803418135 0.00282479813276775 0.00133799988507366;0.00132951476746136 0.00133799988507366 0.00282448912315926]  Capacitance=[7.89543174552926e-09 -1.85986777702161e-09 -1.7901190036642e-09;-1.85986777702161e-09 7.82540023894543e-09 -1.8957321828871e-09;-1.7901190036642e-09 -1.8957321828871e-09 7.91264394645417e-09]  x1=[130.344855189469 9935.82252110572 9935.20612774522;314.159265358979 314.159265358979 314.159265358979;1.02016509751755 -0.184659512344021 -1.75557115185724]  x2=[130.34531972306 9935.75622455115 9935.139980731;314.159265358979 314.159265358979 314.159265358979;1.02016619183365 -0.184660193688182 -1.75557181259691]  x3=[0.114893583406528 24.8704054506803 25.0628110550977;314.159265358979 314.159265358979 314.159265358979;1.01048688893656 -0.174299138354962 -1.74529541026071]  x4=[0.113027529091263 25.6928769463532 25.8855442499484;314.159265358979 314.159265358979 314.159265358979;1.02973100285184 -0.194900714687724 -1.76573298197374]  x5=8.62465088270006e-07  V1=[104.4 5033 5037;314.2 314.2 314.2;0.3469 -0.9264 -2.497]  V2=[104.4 5033 5037;314.2 314.2 314.2;0.3469 -0.9265 -2.497]  I1=[0.0923 12.34 12.45;314.2 314.2 314.2;0.3347 -0.9083 -2.479]  I2=[0.09021 13.28 13.38;314.2 314.2 314.2;0.3591 -0.9435 -2.514]  nHarmo=1  Measurements=None  Decoupling=off  VsMag0=0  VrMag0=0  VsAngle0=0  VrAngle0=0  IsMag0=0  IrMag0=0  IsAngle0=0  IrAngle0=0
      settings: SourceProductBaseCode=PS
  Line 33 : spsDistributedParametersLineLib/Distributed Parameters Line  Phases=3  Length=4.6  Frequency=50  Resistance=[0.646656091154803 0.0486237908083191 0.0486712220507153;0.0486237908083191 0.646561225344642 0.0486237934466192;0.0486712220507153 0.0486237934466192 0.646656091154803]  Inductance=[0.00282448912315926 0.00133270803418135 0.00132951476746136;0.00133270803418135 0.00282479813276775 0.00133799988507366;0.00132951476746136 0.00133799988507366 0.00282448912315926]  Capacitance=[7.89543174552926e-09 -1.85986777702161e-09 -1.7901190036642e-09;-1.85986777702161e-09 7.82540023894543e-09 -1.8957321828871e-09;-1.7901190036642e-09 -1.8957321828871e-09 7.91264394645417e-09]  x1=[130.344855189469 9935.82252110572 9935.20612774522;314.159265358979 314.159265358979 314.159265358979;1.01351173539812 -0.189945171568321 -1.76086184265484]  x2=[130.347980011557 9935.97285079545 9935.35673441657;314.159265358979 314.159265358979 314.159265358979;1.01350139684026 -0.18996442185846 -1.76088125581964]  x3=[0.113712870802751 25.1536156916742 25.3442406042394;314.159265358979 314.159265358979 314.159265358979;1.00658225247795 -0.195455709173532 -1.7663776981781]  x4=[0.113712872834847 25.1536163564059 25.3442412803087;314.159265358979 314.159265358979 314.159265358979;1.01350139684236 -0.189964421858562 -1.76088125581957]  x5=2.20407744780113e-05  V1=[104.4 5033 5037;314.2 314.2 314.2;0.3402 -0.9317 -2.502]  V2=[104.4 5034 5037;314.2 314.2 314.2;0.3402 -0.9318 -2.502]  I1=[0.09105 12.74 12.85;314.2 314.2 314.2;0.3333 -0.9372 -2.507]  I2=[0.09105 12.74 12.85;314.2 314.2 314.2;0.3402 -0.9318 -2.502]  nHarmo=1  Measurements=None  Decoupling=off  VsMag0=0  VrMag0=0  VsAngle0=0  VrAngle0=0  IsMag0=0  IrMag0=0  IsAngle0=0  IrAngle0=0
      settings: SourceProductBaseCode=PS
  Line 34 : spsDistributedParametersLineLib/Distributed Parameters Line  Phases=3  Length=0.35  Frequency=50  Resistance=[0.646656091154803 0.0486237908083191 0.0486712220507153;0.0486237908083191 0.646561225344642 0.0486237934466192;0.0486712220507153 0.0486237934466192 0.646656091154803]  Inductance=[0.00282448912315926 0.00133270803418135 0.00132951476746136;0.00133270803418135 0.00282479813276775 0.00133799988507366;0.00132951476746136 0.00133799988507366 0.00282448912315926]  Capacitance=[7.89543174552926e-09 -1.85986777702161e-09 -1.7901190036642e-09;-1.85986777702161e-09 7.82540023894543e-09 -1.8957321828871e-09;-1.7901190036642e-09 -1.8957321828871e-09 7.91264394645417e-09]  x1=[130.326576288672 9938.31082064819 9937.70046419945;314.159265358979 314.159265358979 314.159265358979;1.01970088187677 -0.184306705852292 -1.75522007120294]  x2=[130.323295421217 9936.32497047719 9935.72733808313;314.159265358979 314.159265358979 314.159265358979;1.01982092712023 -0.184356958602805 -1.7552693847048]  x3=[0.134569186348829 18.5242680498684 18.7418893371848;314.159265358979 314.159265358979 314.159265358979;1.12393651603349 -0.0145456778637025 -1.58830004166616]  x4=[0.095061375881043 32.4529907657693 32.6123868691606;314.159265358979 314.159265358979 314.159265358979;0.871380848215864 -0.281259103368888 -1.85121501390617]  x5=1.6770154494139e-06  V1=[104.3 5037 5041;314.2 314.2 314.2;0.3465 -0.9259 -2.496]  V2=[104.3 5036 5039;314.2 314.2 314.2;0.3466 -0.926 -2.496]  I1=[0.103 6.978 7.072;314.2 314.2 314.2;0.2231 -0.4579 -2.033]  I2=[0.08118 19.65 19.77;314.2 314.2 314.2;0.5028 -1.087 -2.657]  nHarmo=1  Measurements=None  Decoupling=off  VsMag0=0  VrMag0=0  VsAngle0=0  VrAngle0=0  IsMag0=0  IrMag0=0  IsAngle0=0  IrAngle0=0
      settings: SourceProductBaseCode=PS
  Line 35 : spsDistributedParametersLineLib/Distributed Parameters Line  Phases=3  Length=0.09  Frequency=50  Resistance=[0.646656091154803 0.0486237908083191 0.0486712220507153;0.0486237908083191 0.646561225344642 0.0486237934466192;0.0486712220507153 0.0486237934466192 0.646656091154803]  Inductance=[0.00282448912315926 0.00133270803418135 0.00132951476746136;0.00133270803418135 0.00282479813276775 0.00133799988507366;0.00132951476746136 0.00133799988507366 0.00282448912315926]  Capacitance=[7.89543174552926e-09 -1.85986777702161e-09 -1.7901190036642e-09;-1.85986777702161e-09 7.82540023894543e-09 -1.8957321828871e-09;-1.7901190036642e-09 -1.8957321828871e-09 7.91264394645417e-09]  x1=[130.323295421213 9936.32497047662 9935.72733808256;314.159265358979 314.159265358979 314.159265358979;1.02021230136262 -0.184046037471978 -1.75495816759907]  x2=[130.322220657599 9936.00056310743 9935.40495442851;314.159265358979 314.159265358979 314.159265358979;1.02023474989973 -0.184057390408177 -1.7549691667837]  x3=[0.127971033990135 20.6039797125571 20.8341575897062;314.159265358979 314.159265358979 314.159265358979;1.11966637983625 -0.104764408011881 -1.67599214162062]  x4=[0.101344157952782 30.0729022464667 30.228623489466;314.159265358979 314.159265358979 314.159265358979;0.89437595288886 -0.238434568483828 -1.8094535853078]  x5=4.31232544135003e-07  V1=[104.3 5036 5039;314.2 314.2 314.2;0.347 -0.9257 -2.496]  V2=[104.3 5035 5039;314.2 314.2 314.2;0.347 -0.9257 -2.496]  I1=[0.0997 8.795 8.897;314.2 314.2 314.2;0.2278 -0.6939 -2.265]  I2=[0.08427 17.19 17.3;314.2 314.2 314.2;0.488 -1.044 -2.614]  nHarmo=1  Measurements=None  Decoupling=off  VsMag0=0  VrMag0=0  VsAngle0=0  VrAngle0=0  IsMag0=0  IrMag0=0  IsAngle0=0  IrAngle0=0
      settings: SourceProductBaseCode=PS
  Line 36 : spsDistributedParametersLineLib/Distributed Parameters Line  Phases=3  Length=0.32  Frequency=50  Resistance=[0.502970710632245 0.0486237908083191 0.0486712220507153;0.0486237908083191 0.502875844822084 0.0486237934466192;0.0486712220507153 0.0486237934466192 0.502970710632245]  Inductance=[0.00286900545038753 0.00133270803418135 0.00132951476746136;0.00133270803418135 0.00286931445999602 0.00133799988507366;0.00132951476746136 0.00133799988507366 0.00286900545038753]  Capacitance=[8.11484299003193e-09 -1.94249816214699e-09 -1.86930692621136e-09;-1.94249816214699e-09 8.0425699231653e-09 -1.98049571960044e-09;-1.86930692621136e-09 -1.98049571960044e-09 8.13337738722527e-09]  x1=[235.233219494447 9935.96020475674 9935.23346757305;314.159265358979 314.159265358979 314.159265358979;1.00013614296757 -0.178113856899978 -1.74905220304091]  x2=[235.220616169555 9935.0165834557 9934.2954362593;314.159265358979 314.159265358979 314.159265358979;1.0001373791703 -0.178163820795317 -1.74910096060686]  x3=[0.20079451640013 20.6128024060904 20.8427305543518;314.159265358979 314.159265358979 314.159265358979;1.10189996261974 -0.0987246204177554 -1.67003278882865]  x4=[0.213800531690941 30.0792618938501 30.2347267491566;314.159265358979 314.159265358979 314.159265358979;0.904111704066198 -0.232861693557457 -1.80386992116047]  x5=1.54959568730346e-06  V1=[157.3 5035 5038;314.2 314.2 314.2;0.3089 -0.9198 -2.49]  V2=[157.3 5034 5037;314.2 314.2 314.2;0.3088 -0.9198 -2.49]  I1=[0.1289 8.799 8.901;314.2 314.2 314.2;0.2954 -0.688 -2.259]  I2=[0.147 17.19 17.3;314.2 314.2 314.2;0.3202 -1.038 -2.608]  nHarmo=1  Measurements=None  Decoupling=off  VsMag0=0  VrMag0=0  VsAngle0=0  VrAngle0=0  IsMag0=0  IrMag0=0  IsAngle0=0  IrAngle0=0
      settings: SourceProductBaseCode=PS
  Line 37 : spsDistributedParametersLineLib/Distributed Parameters Line  Phases=3  Length=0.06  Frequency=50  Resistance=[0.646656091154803 0.0486237908083191 0.0486712220507153;0.0486237908083191 0.646561225344642 0.0486237934466192;0.0486712220507153 0.0486237934466192 0.646656091154803]  Inductance=[0.00282448912315926 0.00133270803418135 0.00132951476746136;0.00133270803418135 0.00282479813276775 0.00133799988507366;0.00132951476746136 0.00133799988507366 0.00282448912315926]  Capacitance=[7.89543174552926e-09 -1.85986777702161e-09 -1.7901190036642e-09;-1.85986777702161e-09 7.82540023894543e-09 -1.8957321828871e-09;-1.7901190036642e-09 -1.8957321828871e-09 7.91264394645417e-09]  x1=[130.319812743676 9935.05700078356 9934.46688422231;314.159265358979 314.159265358979 314.159265358979;1.02031991867468 -0.184071479946532 -1.75498200847524]  x2=[130.320025715006 9935.02606570402 9934.43601563352;314.159265358979 314.159265358979 314.159265358979;1.02032048850621 -0.184071887141886 -1.75498240574522]  x3=[0.115305192826058 24.6965168335212 24.8889672755871;314.159265358979 314.159265358979 314.159265358979;1.00746567559405 -0.16996596978821 -1.74099094521978]  x4=[0.11259382059821 25.872027906881 26.0648431901396;314.159265358979 314.159265358979 314.159265358979;1.03339289302425 -0.197606578396806 -1.76841243660989]  x5=2.87488362756669e-07  V1=[104.3 5034 5038;314.2 314.2 314.2;0.347 -0.9257 -2.496]  V2=[104.3 5034 5038;314.2 314.2 314.2;0.347 -0.9257 -2.496]  I1=[0.09228 12.35 12.45;314.2 314.2 314.2;0.335 -0.9075 -2.478]  I2=[0.09019 13.28 13.39;314.2 314.2 314.2;0.3592 -0.9428 -2.513]  nHarmo=1  Measurements=None  Decoupling=off  VsMag0=0  VrMag0=0  VsAngle0=0  VrAngle0=0  IsMag0=0  IrMag0=0  IsAngle0=0  IrAngle0=0
      settings: SourceProductBaseCode=PS
  Line 38 : spsDistributedParametersLineLib/Distributed Parameters Line  Phases=3  Length=0.2  Frequency=50  Resistance=[0.502970710632245 0.0486237908083191 0.0486712220507153;0.0486237908083191 0.502875844822084 0.0486237934466192;0.0486712220507153 0.0486237934466192 0.502970710632245]  Inductance=[0.00286900545038753 0.00133270803418135 0.00132951476746136;0.00133270803418135 0.00286931445999602 0.00133799988507366;0.00132951476746136 0.00133799988507366 0.00286900545038753]  Capacitance=[8.11484299003193e-09 -1.94249816214699e-09 -1.86930692621136e-09;-1.94249816214699e-09 8.0425699231653e-09 -1.98049571960044e-09;-1.86930692621136e-09 -1.98049571960044e-09 8.13337738722527e-09]  x1=[235.220616169555 9935.0165834557 9934.2954362593;314.159265358979 314.159265358979 314.159265358979;1.00031993661132 -0.178015972785522 -1.74895294621058]  x2=[235.212859084742 9934.51316337529 9933.79527505067;314.159265358979 314.159265358979 314.159265358979;1.00032227366353 -0.178044589899165 -1.7489808413209]  x3=[0.20184579136577 21.1751857933745 21.4054613025932;314.159265358979 314.159265358979 314.159265358979;1.10173916259699 -0.116763766105044 -1.68785260714438]  x4=[0.212754125631944 29.4769999018705 29.6322920273474;314.159265358979 314.159265358979 314.159265358979;0.903823102005434 -0.222240189086003 -1.79331321297215]  x5=9.68497304564665e-07  V1=[157.3 5034 5037;314.2 314.2 314.2;0.309 -0.9197 -2.49]  V2=[157.3 5034 5037;314.2 314.2 314.2;0.309 -0.9197 -2.49]  I1=[0.1297 9.207 9.31;314.2 314.2 314.2;0.296 -0.7228 -2.294]  I2=[0.1462 16.7 16.81;314.2 314.2 314.2;0.3203 -1.028 -2.598]  nHarmo=1  Measurements=None  Decoupling=off  VsMag0=0  VrMag0=0  VsAngle0=0  VrAngle0=0  IsMag0=0  IrMag0=0  IsAngle0=0  IrAngle0=0
      settings: SourceProductBaseCode=PS
  Line 39 : spsDistributedParametersLineLib/Distributed Parameters Line  Phases=3  Length=0.29  Frequency=50  Resistance=[0.646656091154803 0.0486237908083191 0.0486712220507153;0.0486237908083191 0.646561225344642 0.0486237934466192;0.0486712220507153 0.0486237934466192 0.646656091154803]  Inductance=[0.00282448912315926 0.00133270803418135 0.00132951476746136;0.00133270803418135 0.00282479813276775 0.00133799988507366;0.00132951476746136 0.00133799988507366 0.00282448912315926]  Capacitance=[7.89543174552926e-09 -1.85986777702161e-09 -1.7901190036642e-09;-1.85986777702161e-09 7.82540023894543e-09 -1.8957321828871e-09;-1.7901190036642e-09 -1.8957321828871e-09 7.91264394645417e-09]  x1=[130.317512116336 9934.5536150815 9933.96669495544;314.159265358979 314.159265358979 314.159265358979;1.01999974916509 -0.184375143572145 -1.75528520709046]  x2=[130.323471184292 9933.66136247634 9933.07577650649;314.159265358979 314.159265358979 314.159265358979;1.02002727946395 -0.184408616168706 -1.75531834513707]  x3=[0.124547834262197 21.2025496216257 21.3936967728926;314.159265358979 314.159265358979 314.159265358979;0.959947713619343 -0.122544571881028 -1.69407140637104]  x4=[0.103798165816395 29.4132855621536 29.6065289885366;314.159265358979 314.159265358979 314.159265358979;1.09162541423117 -0.229259121337587 -1.79983255974311]  x5=1.38952708665723e-06  V1=[104.3 5034 5037;314.2 314.2 314.2;0.3466 -0.926 -2.496]  V2=[104.4 5033 5036;314.2 314.2 314.2;0.3467 -0.9261 -2.496]  I1=[0.1002 9.196 9.297;314.2 314.2 314.2;0.2556 -0.7274 -2.3]  I2=[0.08321 16.69 16.8;314.2 314.2 314.2;0.4559 -1.035 -2.605]  nHarmo=1  Measurements=None  Decoupling=off  VsMag0=0  VrMag0=0  VsAngle0=0  VrAngle0=0  IsMag0=0  IrMag0=0  IsAngle0=0  IrAngle0=0
      settings: SourceProductBaseCode=PS
  Line 4 : spsDistributedParametersLineLib/Distributed Parameters Line  Phases=3  Length=0.53  Frequency=50  Resistance=[0.502970710632245 0.0486237908083191 0.0486712220507153;0.0486237908083191 0.502875844822084 0.0486237934466192;0.0486712220507153 0.0486237934466192 0.502970710632245]  Inductance=[0.00286900545038753 0.00133270803418135 0.00132951476746136;0.00133270803418135 0.00286931445999602 0.00133799988507366;0.00132951476746136 0.00133799988507366 0.00286900545038753]  Capacitance=[8.11484299003193e-09 -1.94249816214699e-09 -1.86930692621136e-09;-1.94249816214699e-09 8.0425699231653e-09 -1.98049571960044e-09;-1.86930692621136e-09 -1.98049571960044e-09 8.13337738722527e-09]  x1=[235.499919862763 9971.07620664183 9970.17375086974;314.159265358979 314.159265358979 314.159265358979;1.000055702383 -0.175320495930226 -1.74628341829718]  x2=[235.499801510156 9970.47973890245 9969.57826412568;314.159265358979 314.159265358979 314.159265358979;1.00004238600474 -0.17536142164666 -1.74632404394123]  x3=[0.203423218459154 23.375209957115 23.5674577409211;314.159265358979 314.159265358979 314.159265358979;0.995039906301955 -0.156750866765356 -1.72790596076893]  x4=[0.209596931224635 27.3850342819617 27.5779539308438;314.159265358979 314.159265358979 314.159265358979;1.00411616033149 -0.191814035005515 -1.76263206070293]  x5=2.56651785709636e-06  V1=[157.3 5078 5081;314.2 314.2 314.2;0.31 -0.9152 -2.485]  V2=[157.3 5077 5080;314.2 314.2 314.2;0.31 -0.9152 -2.486]  I1=[0.1333 10.2 10.3;314.2 314.2 314.2;0.305 -0.7979 -2.369]  I2=[0.1426 15.76 15.87;314.2 314.2 314.2;0.3139 -0.9915 -2.561]  nHarmo=1  Measurements=None  Decoupling=off  VsMag0=0  VrMag0=0  VsAngle0=0  VrAngle0=0  IsMag0=0  IrMag0=0  IsAngle0=0  IrAngle0=0
      settings: SourceProductBaseCode=PS
  Line 40 : spsDistributedParametersLineLib/Distributed Parameters Line  Phases=3  Length=0.57  Frequency=50  Resistance=[0.646656091154803 0.0486237908083191 0.0486712220507153;0.0486237908083191 0.646561225344642 0.0486237934466192;0.0486712220507153 0.0486237934466192 0.646656091154803]  Inductance=[0.00282448912315926 0.00133270803418135 0.00132951476746136;0.00133270803418135 0.00282479813276775 0.00133799988507366;0.00132951476746136 0.00133799988507366 0.00282448912315926]  Capacitance=[7.89543174552926e-09 -1.85986777702161e-09 -1.7901190036642e-09;-1.85986777702161e-09 7.82540023894543e-09 -1.8957321828871e-09;-1.7901190036642e-09 -1.8957321828871e-09 7.91264394645417e-09]  x1=[130.323471184292 9933.66136247634 9933.07577650649;314.159265358979 314.159265358979 314.159265358979;1.01960579951068 -0.184743454309612 -1.75565350202018]  x2=[130.328621629531 9932.92517766288 9932.34124789717;314.159265358979 314.159265358979 314.159265358979;1.0196179978007 -0.184751021699709 -1.7556608402866]  x3=[0.117252946643836 23.8388948559524 24.0306953449004;314.159265358979 314.159265358979 314.159265358979;0.986470712555958 -0.14680453435418 -1.71803548771297]  x4=[0.110710245793674 26.7195672227095 26.9123080044511;314.159265358979 314.159265358979 314.159265358979;1.05382895145188 -0.219242615444824 -1.78989479055827]  x5=2.73113944618835e-06  V1=[104.4 5033 5036;314.2 314.2 314.2;0.3462 -0.9264 -2.497]  V2=[104.4 5032 5036;314.2 314.2 314.2;0.3462 -0.9264 -2.497]  I1=[0.09388 11.65 11.75;314.2 314.2 314.2;0.3162 -0.8786 -2.449]  I2=[0.08864 13.98 14.08;314.2 314.2 314.2;0.3772 -0.9669 -2.537]  nHarmo=1  Measurements=None  Decoupling=off  VsMag0=0  VrMag0=0  VsAngle0=0  VrAngle0=0  IsMag0=0  IrMag0=0  IsAngle0=0  IrAngle0=0
      settings: SourceProductBaseCode=PS
  Line 41 : spsDistributedParametersLineLib/Distributed Parameters Line  Phases=3  Length=0.17  Frequency=50  Resistance=[0.646656091154803 0.0486237908083191 0.0486712220507153;0.0486237908083191 0.646561225344642 0.0486237934466192;0.0486712220507153 0.0486237934466192 0.646656091154803]  Inductance=[0.00282448912315926 0.00133270803418135 0.00132951476746136;0.00133270803418135 0.00282479813276775 0.00133799988507366;0.00132951476746136 0.00133799988507366 0.00282448912315926]  Capacitance=[7.89543174552926e-09 -1.85986777702161e-09 -1.7901190036642e-09;-1.85986777702161e-09 7.82540023894543e-09 -1.8957321828871e-09;-1.7901190036642e-09 -1.8957321828871e-09 7.91264394645417e-09]  x1=[130.323471184292 9933.66136247634 9933.07577650649;314.159265358979 314.159265358979 314.159265358979;1.02020791372963 -0.184265114108318 -1.75517470647288]  x2=[130.325402522049 9933.35664285287 9932.77134263119;314.159265358979 314.159265358979 314.159265358979;1.02022049857711 -0.184282322197882 -1.75519178540436]  x3=[0.121112900449845 22.6089418961166 22.8009875996086;314.159265358979 314.159265358979 314.159265358979;0.990968907364386 -0.165935113439156 -1.73703649787403]  x4=[0.106872182076276 27.9475847084714 28.1406311239185;314.159265358979 314.159265358979 314.159265358979;1.05308481180397 -0.199292817190908 -1.77007058732592]  x5=8.14550361143895e-07  V1=[104.4 5033 5036;314.2 314.2 314.2;0.3468 -0.9259 -2.496]  V2=[104.4 5032 5036;314.2 314.2 314.2;0.3468 -0.926 -2.496]  I1=[0.09733 10.26 10.36;314.2 314.2 314.2;0.2826 -0.8025 -2.374]  I2=[0.08557 15.48 15.59;314.2 314.2 314.2;0.4197 -1.008 -2.577]  nHarmo=1  Measurements=None  Decoupling=off  VsMag0=0  VrMag0=0  VsAngle0=0  VrAngle0=0  IsMag0=0  IrMag0=0  IsAngle0=0  IrAngle0=0
      settings: SourceProductBaseCode=PS
  Line 42 : spsDistributedParametersLineLib/Distributed Parameters Line  Phases=3  Length=0.01  Frequency=50  Resistance=[0.502970710632245 0.0486237908083191 0.0486712220507153;0.0486237908083191 0.502875844822084 0.0486237934466192;0.0486712220507153 0.0486237934466192 0.502970710632245]  Inductance=[0.00286900545038753 0.00133270803418135 0.00132951476746136;0.00133270803418135 0.00286931445999602 0.00133799988507366;0.00132951476746136 0.00133799988507366 0.00286900545038753]  Capacitance=[8.11484299003193e-09 -1.94249816214699e-09 -1.86930692621136e-09;-1.94249816214699e-09 8.0425699231653e-09 -1.98049571960044e-09;-1.86930692621136e-09 -1.98049571960044e-09 8.13337738722527e-09]  x1=[235.207859983321 9933.31617141168 9932.59987080656;314.159265358979 314.159265358979 314.159265358979;1.00061310761344 -0.177861181389975 -1.74879670407931]  x2=[235.207856433976 9933.31005798999 9932.59376756515;314.159265358979 314.159265358979 314.159265358979;1.00061297614079 -0.177861579607609 -1.74879709924655]  x3=[0.204638379271632 24.2287222652699 24.4210449060733;314.159265358979 314.159265358979 314.159265358979;0.998811603119193 -0.16698298707133 -1.738019798401]  x4=[0.207950527299813 26.3586308370497 26.551369650621;314.159265358979 314.159265358979 314.159265358979;1.0023706980735 -0.187872537866423 -1.75872112407423]  x5=4.84248652282332e-08  V1=[157.3 5032 5036;314.2 314.2 314.2;0.3093 -0.9195 -2.49]  V2=[157.3 5032 5036;314.2 314.2 314.2;0.3093 -0.9195 -2.49]  I1=[0.136 11.66 11.77;314.2 314.2 314.2;0.3099 -0.8711 -2.442]  I2=[0.14 13.99 14.1;314.2 314.2 314.2;0.3087 -0.96 -2.53]  nHarmo=1  Measurements=None  Decoupling=off  VsMag0=0  VrMag0=0  VsAngle0=0  VrAngle0=0  IsMag0=0  IrMag0=0  IsAngle0=0  IrAngle0=0
      settings: SourceProductBaseCode=PS
  Line 43 : spsDistributedParametersLineLib/Distributed Parameters Line  Phases=3  Length=0.41001  Frequency=50  Resistance=[0.646656091154803 0.0486237908083191 0.0486712220507153;0.0486237908083191 0.646561225344642 0.0486237934466192;0.0486712220507153 0.0486237934466192 0.646656091154803]  Inductance=[0.00282448912315926 0.00133270803418135 0.00132951476746136;0.00133270803418135 0.00282479813276775 0.00133799988507366;0.00132951476746136 0.00133799988507366 0.00282448912315926]  Capacitance=[7.89543174552926e-09 -1.85986777702161e-09 -1.7901190036642e-09;-1.85986777702161e-09 7.82540023894543e-09 -1.8957321828871e-09;-1.7901190036642e-09 -1.8957321828871e-09 7.91264394645417e-09]  x1=[130.325402522049 9933.35664285287 9932.77134263119;314.159265358979 314.159265358979 314.159265358979;1.01985921499289 -0.184569338277164 -1.75547907470263]  x2=[130.328033165372 9932.93187309652 9932.34687726225;314.159265358979 314.159265358979 314.159265358979;1.01987851256563 -0.184596472666679 -1.75550602073803]  x3=[0.118299011068912 23.6631519037667 23.8553532616568;314.159265358979 314.159265358979 314.159265358979;1.0039527444382 -0.177977234879395 -1.74896269744992]  x4=[0.10958388594217 26.8717690920743 27.064504056566;314.159265358979 314.159265358979 314.159265358979;1.03640912677671 -0.190860926251139 -1.76170986894415]  x5=1.9645517268977e-06  V1=[104.4 5032 5036;314.2 314.2 314.2;0.3465 -0.9262 -2.496]  V2=[104.4 5032 5035;314.2 314.2 314.2;0.3465 -0.9263 -2.496]  I1=[0.09456 11.36 11.47;314.2 314.2 314.2;0.3096 -0.8646 -2.435]  I2=[0.08802 14.28 14.38;314.2 314.2 314.2;0.3854 -0.9758 -2.546]  nHarmo=1  Measurements=None  Decoupling=off  VsMag0=0  VrMag0=0  VsAngle0=0  VrAngle0=0  IsMag0=0  IrMag0=0  IsAngle0=0  IrAngle0=0
      settings: SourceProductBaseCode=PS
  Line 5 : spsDistributedParametersLineLib/Distributed Parameters Line  Phases=3  Length=0.26  Frequency=50  Resistance=[0.502970710632245 0.0486237908083191 0.0486712220507153;0.0486237908083191 0.502875844822084 0.0486237934466192;0.0486712220507153 0.0486237934466192 0.502970710632245]  Inductance=[0.00286900545038753 0.00133270803418135 0.00132951476746136;0.00133270803418135 0.00286931445999602 0.00133799988507366;0.00132951476746136 0.00133799988507366 0.00286900545038753]  Capacitance=[8.11484299003193e-09 -1.94249816214699e-09 -1.86930692621136e-09;-1.94249816214699e-09 8.0425699231653e-09 -1.98049571960044e-09;-1.86930692621136e-09 -1.98049571960044e-09 8.13337738722527e-09]  x1=[235.499801510156 9970.47973890245 9969.57826412568;314.159265358979 314.159265358979 314.159265358979;1.00045314024704 -0.175028763624621 -1.74599101154961]  x2=[235.499516587529 9970.30560160173 9969.40459248384;314.159265358979 314.159265358979 314.159265358979;1.00045007127819 -0.17503396072491 -1.74599614315181]  x3=[0.204903122340889 24.4775793539571 24.6699646135071;314.159265358979 314.159265358979 314.159265358979;1.00059623422033 -0.153531882903647 -1.72467694893725]  x4=[0.208156346290404 26.2959219048241 26.4888646604629;314.159265358979 314.159265358979 314.159265358979;0.999916774070504 -0.195353243674547 -1.76615597224583]  x5=1.25904649593406e-06  V1=[157.3 5077 5080;314.2 314.2 314.2;0.3104 -0.9149 -2.485]  V2=[157.3 5076 5079;314.2 314.2 314.2;0.3104 -0.9149 -2.485]  I1=[0.1348 11.11 11.21;314.2 314.2 314.2;0.3109 -0.8343 -2.405]  I2=[0.1411 14.8 14.91;314.2 314.2 314.2;0.3096 -0.9756 -2.545]  nHarmo=1  Measurements=None  Decoupling=off  VsMag0=0  VrMag0=0  VsAngle0=0  VrAngle0=0  IsMag0=0  IrMag0=0  IsAngle0=0  IrAngle0=0
      settings: SourceProductBaseCode=PS
  Line 6 : spsDistributedParametersLineLib/Distributed Parameters Line  Phases=3  Length=0.06  Frequency=50  Resistance=[0.502970710632245 0.0486237908083191 0.0486712220507153;0.0486237908083191 0.502875844822084 0.0486237934466192;0.0486712220507153 0.0486237934466192 0.502970710632245]  Inductance=[0.00286900545038753 0.00133270803418135 0.00132951476746136;0.00133270803418135 0.00286931445999602 0.00133799988507366;0.00132951476746136 0.00133799988507366 0.00286900545038753]  Capacitance=[8.11484299003193e-09 -1.94249816214699e-09 -1.86930692621136e-09;-1.94249816214699e-09 8.0425699231653e-09 -1.98049571960044e-09;-1.86930692621136e-09 -1.98049571960044e-09 8.13337738722527e-09]  x1=[235.499801510156 9970.47973890245 9969.57826412568;314.159265358979 314.159265358979 314.159265358979;1.00075740264875 -0.174782350274962 -1.74574432088915]  x2=[235.499839967303 9970.45201486549 9969.55054283553;314.159265358979 314.159265358979 314.159265358979;1.0007566237301 -0.174785748016908 -1.74574769945977]  x3=[0.205087131414315 24.2891728933869 24.4818924889057;314.159265358979 314.159265358979 314.159265358979;0.996450559246237 -0.177892976395619 -1.74884840240267]  x4=[0.208008827725689 26.482641022852 26.6754830008782;314.159265358979 314.159265358979 314.159265358979;1.00491234016225 -0.172003488381165 -1.74296970151393]  x5=2.90549191369399e-07  V1=[157.3 5077 5080;314.2 314.2 314.2;0.3107 -0.9147 -2.485]  V2=[157.3 5077 5080;314.2 314.2 314.2;0.3107 -0.9147 -2.485]  I1=[0.1365 11.99 12.09;314.2 314.2 314.2;0.3061 -0.889 -2.46]  I2=[0.1394 13.87 13.98;314.2 314.2 314.2;0.3151 -0.9369 -2.507]  nHarmo=1  Measurements=None  Decoupling=off  VsMag0=0  VrMag0=0  VsAngle0=0  VrAngle0=0  IsMag0=0  IrMag0=0  IsAngle0=0  IrAngle0=0
      settings: SourceProductBaseCode=PS
  Line 7 : spsDistributedParametersLineLib/Distributed Parameters Line  Phases=3  Length=0.13  Frequency=50  Resistance=[0.476003738225748 0.351747138225748 0.351747138225748;0.351747138225748 0.476003738225748 0.351747138225748;0.351747138225748 0.351747138225748 0.476003738225748]  Inductance=[0.000705954362986426 0.000459934243504405 0.000459934243504405;0.000459934243504405 0.000705954362986426 0.000459934243504405;0.000459934243504405 0.000459934243504405 0.000705954362986426]  Capacitance=[5.7561313269996e-07 -1.37543883484145e-07 -1.37543912800485e-07;-1.37543883484145e-07 5.75613027339387e-07 -1.37543875208088e-07;-1.37543912800485e-07 -1.37543875208088e-07 5.75613005057695e-07]  x1=[0.598445586093793 9971.51860753636 9971.67511878749;314.159265358979 314.159265358979 314.159265358979;1.74988029451972 -0.099836535191671 -1.67061633456104]  x2=[0.598445831830563 9971.50017588966 9971.65668685126;314.159265358979 314.159265358979 314.159265358979;1.74987936058545 -0.0998375247071843 -1.67061732407651]  x3=[0.00812364329287977 535.423038235277 535.431400694323;314.159265358979 314.159265358979 314.159265358979;1.74897937358465 -0.099974484391599 -1.67075428368597]  x4=[0.00812360271751454 537.614489065983 537.622885921332;314.159265358979 314.159265358979 314.159265358979;1.7498770654022 -0.100240118048813 -1.67101991745086]  x5=2.87356129084973e-06  V1=[38.27 5077 5081;314.2 314.2 314.2;0.4695 -0.8397 -2.41]  V2=[38.27 5077 5081;314.2 314.2 314.2;0.4695 -0.8397 -2.41]  I1=[0.5195 272.2 272.5;314.2 314.2 314.2;0.4686 -0.8385 -2.409]  I2=[0.5195 274.1 274.3;314.2 314.2 314.2;0.4695 -0.8413 -2.412]  nHarmo=1  Measurements=None  Decoupling=off  VsMag0=0  VrMag0=0  VsAngle0=0  VrAngle0=0  IsMag0=0  IrMag0=0  IsAngle0=0  IrAngle0=0
      settings: SourceProductBaseCode=PS
  Line 8 : spsDistributedParametersLineLib/Distributed Parameters Line  Phases=3  Length=1.19  Frequency=50  Resistance=[0.502970710632245 0.0486237908083191 0.0486712220507153;0.0486237908083191 0.502875844822084 0.0486237934466192;0.0486712220507153 0.0486237934466192 0.502970710632245]  Inductance=[0.00286900545038753 0.00133270803418135 0.00132951476746136;0.00133270803418135 0.00286931445999602 0.00133799988507366;0.00132951476746136 0.00133799988507366 0.00286900545038753]  Capacitance=[8.11484299003193e-09 -1.94249816214699e-09 -1.86930692621136e-09;-1.94249816214699e-09 8.0425699231653e-09 -1.98049571960044e-09;-1.86930692621136e-09 -1.98049571960044e-09 8.13337738722527e-09]  x1=[235.499919862763 9971.07620664183 9970.17375086974;314.159265358979 314.159265358979 314.159265358979;0.99905163645738 -0.176133659984099 -1.74709749747669]  x2=[235.453514952772 9963.46848629237 9962.60262698438;314.159265358979 314.159265358979 314.159265358979;0.998960819478773 -0.176796753638202 -1.74775546797805]  x3=[0.190999493485675 12.7415617740978 12.9608504687473;314.159265358979 314.159265358979 314.159265358979;1.08660182826358 -0.0754438510745861 -1.65002049974831]  x4=[0.223255283136056 38.0519852361626 38.213018996728;314.159265358979 314.159265358979 314.159265358979;0.922413107037566 -0.211218333146282 -1.7813997412612]  x5=5.76255896215976e-06  V1=[157.3 5078 5081;314.2 314.2 314.2;0.309 -0.916 -2.486]  V2=[157.3 5068 5071;314.2 314.2 314.2;0.3086 -0.9171 -2.487]  I1=[0.1138 4.051 4.043;314.2 314.2 314.2;0.2108 0.8236 -0.7699]  I2=[0.1629 26.79 26.91;314.2 314.2 314.2;0.3758 -1.067 -2.637]  nHarmo=1  Measurements=None  Decoupling=off  VsMag0=0  VrMag0=0  VsAngle0=0  VrAngle0=0  IsMag0=0  IrMag0=0  IsAngle0=0  IrAngle0=0
      settings: SourceProductBaseCode=PS
  Line 9 : spsDistributedParametersLineLib/Distributed Parameters Line  Phases=3  Length=0.01  Frequency=50  Resistance=[0.646656091154803 0.0486237908083191 0.0486712220507153;0.0486237908083191 0.646561225344642 0.0486237934466192;0.0486712220507153 0.0486237934466192 0.646656091154803]  Inductance=[0.00282448912315926 0.00133270803418135 0.00132951476746136;0.00133270803418135 0.00282479813276775 0.00133799988507366;0.00132951476746136 0.00133799988507366 0.00282448912315926]  Capacitance=[7.89543174552926e-09 -1.85986777702161e-09 -1.7901190036642e-09;-1.85986777702161e-09 7.82540023894543e-09 -1.8957321828871e-09;-1.7901190036642e-09 -1.8957321828871e-09 7.91264394645417e-09]  x1=[130.242577399402 9963.50829942501 9962.77347738552;314.159265358979 314.159265358979 314.159265358979;1.01877502615297 -0.18157273583244 -1.75250377764255]  x2=[130.242588853237 9963.5066576949 9962.77183955524;314.159265358979 314.159265358979 314.159265358979;1.01877505019487 -0.181572745052055 -1.75250378636653]  x3=[0.114271430905508 25.1788443784862 25.3716442857688;314.159265358979 314.159265358979 314.159265358979;1.01443725076919 -0.176657396465351 -1.74762726144723]  x4=[0.113480898571888 25.5332480772748 25.7261632073533;314.159265358979 314.159265358979 314.159265358979;1.0231279396025 -0.186431734034999 -1.75732498869965]  x5=4.79147271261115e-08  V1=[104 5068 5071;314.2 314.2 314.2;0.3472 -0.9219 -2.492]  V2=[104 5068 5071;314.2 314.2 314.2;0.3472 -0.9219 -2.492]  I1=[0.09157 12.6 12.71;314.2 314.2 314.2;0.3397 -0.9106 -2.481]  I2=[0.09025 13.19 13.3;314.2 314.2 314.2;0.3549 -0.9326 -2.503]  nHarmo=1  Measurements=None  Decoupling=off  VsMag0=0  VrMag0=0  VsAngle0=0  VrAngle0=0  IsMag0=0  IrMag0=0  IsAngle0=0  IrAngle0=0
      settings: SourceProductBaseCode=PS
  Line im1 : spsDistributedParametersLineLib/Distributed Parameters Line  Phases=3  Length=1e-10  Frequency=50  Resistance=[0.646656091154803 0.0486237908083191 0.0486712220507153;0.0486237908083191 0.646561225344642 0.0486237934466192;0.0486712220507153 0.0486237934466192 0.646656091154803]  Inductance=[0.00282448912315926 0.00133270803418135 0.00132951476746136;0.00133270803418135 0.00282479813276775 0.00133799988507366;0.00132951476746136 0.00133799988507366 0.00282448912315926]  Capacitance=[7.89543174552926e-09 -1.85986777702161e-09 -1.7901190036642e-09;-1.85986777702161e-09 7.82540023894543e-09 -1.8957321828871e-09;-1.7901190036642e-09 -1.8957321828871e-09 7.91264394645417e-09]  x1=[130.323295421217 9936.32497047719 9935.72733808313;314.159265358979 314.159265358979 314.159265358979;1.02034777706166 -0.183938410926792 -1.75485043860103]  x2=[130.323295421213 9936.32497047662 9935.72733808256;314.159265358979 314.159265358979 314.159265358979;1.02034777706174 -0.183938410926807 -1.75485043860105]  x3=[0.160468204516422 18.5042397015992 18.7088632106749;314.159265358979 314.159265358979 314.159265358979;1.39621511277405 -0.0140257685984978 -1.58587314689122]  x4=[0.0822646094138804 32.4894681589693 32.6672911904719;314.159265358979 314.159265358979 314.159265358979;0.544893634987909 -0.280793148091997 -1.85193990244352]  x5=4.79147271261115e-16  V1=[104.3 5036 5039;314.2 314.2 314.2;0.3471 -0.9256 -2.496]  V2=[104.3 5036 5039;314.2 314.2 314.2;0.3471 -0.9256 -2.496]  I1=[0.1149 7.004 7.142;314.2 314.2 314.2;0.4879 -0.4472 -2.04]  I2=[0.06723 19.68 19.68;314.2 314.2 314.2;0.07907 -1.09 -2.656]  nHarmo=1  Measurements=None  Decoupling=off  VsMag0=0  VrMag0=0  VsAngle0=0  VrAngle0=0  IsMag0=0  IrMag0=0  IsAngle0=0  IrAngle0=0
      settings: SourceProductBaseCode=PS
  Line im2 : spsDistributedParametersLineLib/Distributed Parameters Line  Phases=3  Length=1e-10  Frequency=50  Resistance=[0.502970710632245 0.0486237908083191 0.0486712220507153;0.0486237908083191 0.502875844822084 0.0486237934466192;0.0486712220507153 0.0486237934466192 0.502970710632245]  Inductance=[0.00286900545038753 0.00133270803418135 0.00132951476746136;0.00133270803418135 0.00286931445999602 0.00133799988507366;0.00132951476746136 0.00133799988507366 0.00286900545038753]  Capacitance=[8.11484299003193e-09 -1.94249816214699e-09 -1.86930692621136e-09;-1.94249816214699e-09 8.0425699231653e-09 -1.98049571960044e-09;-1.86930692621136e-09 -1.98049571960044e-09 8.13337738722527e-09]  x1=[235.212859084742 9934.51316337529 9933.79527505067;314.159265358979 314.159265358979 314.159265358979;1.00062653606508 -0.17779817654963 -1.74873415066056]  x2=[235.212859084741 9934.51316337529 9933.79527505068;314.159265358979 314.159265358979 314.159265358979;1.00062653606509 -0.17779817654963 -1.74873415066056]  x3=[0.214768621997318 25.2925946093558 25.5818036809496;314.159265358979 314.159265358979 314.159265358979;1.09144397609372 -0.178338492469116 -1.75482449008998]  x4=[0.182754504246437 25.2806937412556 25.3863383356351;314.159265358979 314.159265358979 314.159265358979;0.938636479938896 -0.177378906084441 -1.74268933625103]  x5=4.84248652282332e-16  V1=[157.3 5034 5037;314.2 314.2 314.2;0.3093 -0.9195 -2.49]  V2=[157.3 5034 5037;314.2 314.2 314.2;0.3093 -0.9195 -2.49]  I1=[0.139 12.79 12.95;314.2 314.2 314.2;0.3799 -0.9192 -2.491]  I2=[0.1429 12.83 12.9;314.2 314.2 314.2;0.2608 -0.9199 -2.489]  nHarmo=1  Measurements=None  Decoupling=off  VsMag0=0  VrMag0=0  VsAngle0=0  VrAngle0=0  IsMag0=0  IrMag0=0  IsAngle0=0  IrAngle0=0
      settings: SourceProductBaseCode=PS
  Load 171 : spsThreePhaseSeriesRLCLoadLib/Three-Phase Series RLC Load  LConnTagsString=A|B|C  Configuration=Delta  NominalVoltage=10000  Vabc=[1e3 1e3 1e3]  Vabcp=[1e3 1e3 1e3]  NominalFrequency=50  UnbalancedPower=off  ActivePower=8093.9097  InductivePower=4050.478  CapacitivePower=0  Pabc=[10e3 9e3 11e3]  QLabc=[100 90 110]  QCabc=[100 90 110]  Pabcp=[10e3 9e3 11e3]  QLabcp=[100 90 110]  QCabcp=[100 90 110]  Measurements=None  LoadType=constant Z
  Load 174 : spsThreePhaseSeriesRLCLoadLib/Three-Phase Series RLC Load  LConnTagsString=A|B|C  Configuration=Delta  NominalVoltage=10000  Vabc=[1e3 1e3 1e3]  Vabcp=[1e3 1e3 1e3]  NominalFrequency=50  UnbalancedPower=off  ActivePower=6644.0013  InductivePower=4375.2483  CapacitivePower=0  Pabc=[10e3 9e3 11e3]  QLabc=[100 90 110]  QCabc=[100 90 110]  Pabcp=[10e3 9e3 11e3]  QLabcp=[100 90 110]  QCabcp=[100 90 110]  Measurements=None  LoadType=constant Z
  Load 178 : spsThreePhaseSeriesRLCLoadLib/Three-Phase Series RLC Load  LConnTagsString=A|B|C  Configuration=Delta  NominalVoltage=10000  Vabc=[1e3 1e3 1e3]  Vabcp=[1e3 1e3 1e3]  NominalFrequency=50  UnbalancedPower=off  ActivePower=2397.2302  InductivePower=1196.8054  CapacitivePower=0  Pabc=[10e3 9e3 11e3]  QLabc=[100 90 110]  QCabc=[100 90 110]  Pabcp=[10e3 9e3 11e3]  QLabcp=[100 90 110]  QCabcp=[100 90 110]  Measurements=None  LoadType=constant Z
  Load 1873 : spsThreePhaseSeriesRLCLoadLib/Three-Phase Series RLC Load  LConnTagsString=A|B|C  Configuration=Delta  NominalVoltage=10000  Vabc=[1e3 1e3 1e3]  Vabcp=[1e3 1e3 1e3]  NominalFrequency=50  UnbalancedPower=off  ActivePower=2293.6414  InductivePower=1310.764  CapacitivePower=0  Pabc=[10e3 9e3 11e3]  QLabc=[100 90 110]  QCabc=[100 90 110]  Pabcp=[10e3 9e3 11e3]  QLabcp=[100 90 110]  QCabcp=[100 90 110]  Measurements=None  LoadType=constant Z
  Load 534 : spsThreePhaseSeriesRLCLoadLib/Three-Phase Series RLC Load  LConnTagsString=A|B|C  Configuration=Delta  NominalVoltage=10000  Vabc=[1e3 1e3 1e3]  Vabcp=[1e3 1e3 1e3]  NominalFrequency=50  UnbalancedPower=off  ActivePower=17310.4266  InductivePower=11256.0499  CapacitivePower=0  Pabc=[10e3 9e3 11e3]  QLabc=[100 90 110]  QCabc=[100 90 110]  Pabcp=[10e3 9e3 11e3]  QLabcp=[100 90 110]  QCabcp=[100 90 110]  Measurements=None  LoadType=constant Z
  Load 535 : spsThreePhaseSeriesRLCLoadLib/Three-Phase Series RLC Load  LConnTagsString=A|B|C  Configuration=Delta  NominalVoltage=10000  Vabc=[1e3 1e3 1e3]  Vabcp=[1e3 1e3 1e3]  NominalFrequency=50  UnbalancedPower=off  ActivePower=9735.7818  InductivePower=6070.259  CapacitivePower=0  Pabc=[10e3 9e3 11e3]  QLabc=[100 90 110]  QCabc=[100 90 110]  Pabcp=[10e3 9e3 11e3]  QLabcp=[100 90 110]  QCabcp=[100 90 110]  Measurements=None  LoadType=constant Z
  Load 8042 : spsThreePhaseSeriesRLCLoadLib/Three-Phase Series RLC Load  LConnTagsString=A|B|C  Configuration=Delta  NominalVoltage=10000  Vabc=[1e3 1e3 1e3]  Vabcp=[1e3 1e3 1e3]  NominalFrequency=50  UnbalancedPower=off  ActivePower=1006.297  InductivePower=613.553  CapacitivePower=0  Pabc=[10e3 9e3 11e3]  QLabc=[100 90 110]  QCabc=[100 90 110]  Pabcp=[10e3 9e3 11e3]  QLabcp=[100 90 110]  QCabcp=[100 90 110]  Measurements=None  LoadType=constant Z
  Load 8130 : spsThreePhaseSeriesRLCLoadLib/Three-Phase Series RLC Load  LConnTagsString=A|B|C  Configuration=Delta  NominalVoltage=10000  Vabc=[1e3 1e3 1e3]  Vabcp=[1e3 1e3 1e3]  NominalFrequency=50  UnbalancedPower=off  ActivePower=17862.6645  InductivePower=11643.8869  CapacitivePower=0  Pabc=[10e3 9e3 11e3]  QLabc=[100 90 110]  QCabc=[100 90 110]  Pabcp=[10e3 9e3 11e3]  QLabcp=[100 90 110]  QCabcp=[100 90 110]  Measurements=None  LoadType=constant Z
  Load 8131 : spsThreePhaseSeriesRLCLoadLib/Three-Phase Series RLC Load  LConnTagsString=A|B|C  Configuration=Delta  NominalVoltage=10000  Vabc=[1e3 1e3 1e3]  Vabcp=[1e3 1e3 1e3]  NominalFrequency=50  UnbalancedPower=off  ActivePower=26372.175  InductivePower=18529.6749  CapacitivePower=0  Pabc=[10e3 9e3 11e3]  QLabc=[100 90 110]  QCabc=[100 90 110]  Pabcp=[10e3 9e3 11e3]  QLabcp=[100 90 110]  QCabcp=[100 90 110]  Measurements=None  LoadType=constant Z
  Load 8193 : spsThreePhaseSeriesRLCLoadLib/Three-Phase Series RLC Load  LConnTagsString=A|B|C  Configuration=Delta  NominalVoltage=10000  Vabc=[1e3 1e3 1e3]  Vabcp=[1e3 1e3 1e3]  NominalFrequency=50  UnbalancedPower=off  ActivePower=18613.6873  InductivePower=6959.3447  CapacitivePower=0  Pabc=[10e3 9e3 11e3]  QLabc=[100 90 110]  QCabc=[100 90 110]  Pabcp=[10e3 9e3 11e3]  QLabcp=[100 90 110]  QCabcp=[100 90 110]  Measurements=None  LoadType=constant Z
  Load 8201 : spsThreePhaseSeriesRLCLoadLib/Three-Phase Series RLC Load  LConnTagsString=A|B|C  Configuration=Delta  NominalVoltage=10000  Vabc=[1e3 1e3 1e3]  Vabcp=[1e3 1e3 1e3]  NominalFrequency=50  UnbalancedPower=off  ActivePower=14776.8697  InductivePower=7768.0787  CapacitivePower=0  Pabc=[10e3 9e3 11e3]  QLabc=[100 90 110]  QCabc=[100 90 110]  Pabcp=[10e3 9e3 11e3]  QLabcp=[100 90 110]  QCabcp=[100 90 110]  Measurements=None  LoadType=constant Z
  Load 8202 : spsThreePhaseSeriesRLCLoadLib/Three-Phase Series RLC Load  LConnTagsString=A|B|C  Configuration=Delta  NominalVoltage=10000  Vabc=[1e3 1e3 1e3]  Vabcp=[1e3 1e3 1e3]  NominalFrequency=50  UnbalancedPower=off  ActivePower=16457.0301  InductivePower=6528.8727  CapacitivePower=0  Pabc=[10e3 9e3 11e3]  QLabc=[100 90 110]  QCabc=[100 90 110]  Pabcp=[10e3 9e3 11e3]  QLabcp=[100 90 110]  QCabcp=[100 90 110]  Measurements=None  LoadType=constant Z
  Load 8429 : spsThreePhaseSeriesRLCLoadLib/Three-Phase Series RLC Load  LConnTagsString=A|B|C  Configuration=Delta  NominalVoltage=10000  Vabc=[1e3 1e3 1e3]  Vabcp=[1e3 1e3 1e3]  NominalFrequency=50  UnbalancedPower=off  ActivePower=6691.7956  InductivePower=2704.2118  CapacitivePower=0  Pabc=[10e3 9e3 11e3]  QLabc=[100 90 110]  QCabc=[100 90 110]  Pabcp=[10e3 9e3 11e3]  QLabcp=[100 90 110]  QCabcp=[100 90 110]  Measurements=None  LoadType=constant Z
  Load 8468 : spsThreePhaseSeriesRLCLoadLib/Three-Phase Series RLC Load  LConnTagsString=A|B|C  Configuration=Delta  NominalVoltage=10000  Vabc=[1e3 1e3 1e3]  Vabcp=[1e3 1e3 1e3]  NominalFrequency=50  UnbalancedPower=off  ActivePower=5163.0004  InductivePower=3310.8596  CapacitivePower=0  Pabc=[10e3 9e3 11e3]  QLabc=[100 90 110]  QCabc=[100 90 110]  Pabcp=[10e3 9e3 11e3]  QLabcp=[100 90 110]  QCabcp=[100 90 110]  Measurements=None  LoadType=constant Z
  Load 8478 : spsThreePhaseSeriesRLCLoadLib/Three-Phase Series RLC Load  LConnTagsString=A|B|C  Configuration=Delta  NominalVoltage=10000  Vabc=[1e3 1e3 1e3]  Vabcp=[1e3 1e3 1e3]  NominalFrequency=50  UnbalancedPower=off  ActivePower=6880.5372  InductivePower=4313.9119  CapacitivePower=0  Pabc=[10e3 9e3 11e3]  QLabc=[100 90 110]  QCabc=[100 90 110]  Pabcp=[10e3 9e3 11e3]  QLabcp=[100 90 110]  QCabcp=[100 90 110]  Measurements=None  LoadType=constant Z
  Load 8590 : spsThreePhaseSeriesRLCLoadLib/Three-Phase Series RLC Load  LConnTagsString=A|B|C  Configuration=Delta  NominalVoltage=10000  Vabc=[1e3 1e3 1e3]  Vabcp=[1e3 1e3 1e3]  NominalFrequency=50  UnbalancedPower=off  ActivePower=2956.8776  InductivePower=1246.5667  CapacitivePower=0  Pabc=[10e3 9e3 11e3]  QLabc=[100 90 110]  QCabc=[100 90 110]  Pabcp=[10e3 9e3 11e3]  QLabcp=[100 90 110]  QCabcp=[100 90 110]  Measurements=None  LoadType=constant Z
  Load 8624 : spsThreePhaseSeriesRLCLoadLib/Three-Phase Series RLC Load  LConnTagsString=A|B|C  Configuration=Delta  NominalVoltage=10000  Vabc=[1e3 1e3 1e3]  Vabcp=[1e3 1e3 1e3]  NominalFrequency=50  UnbalancedPower=off  ActivePower=5239.8943  InductivePower=2659.1136  CapacitivePower=0  Pabc=[10e3 9e3 11e3]  QLabc=[100 90 110]  QCabc=[100 90 110]  Pabcp=[10e3 9e3 11e3]  QLabcp=[100 90 110]  QCabcp=[100 90 110]  Measurements=None  LoadType=constant Z
  Load 8693 : spsThreePhaseSeriesRLCLoadLib/Three-Phase Series RLC Load  LConnTagsString=A|B|C  Configuration=Delta  NominalVoltage=10000  Vabc=[1e3 1e3 1e3]  Vabcp=[1e3 1e3 1e3]  NominalFrequency=50  UnbalancedPower=off  ActivePower=17700.7491  InductivePower=5558.9797  CapacitivePower=0  Pabc=[10e3 9e3 11e3]  QLabc=[100 90 110]  QCabc=[100 90 110]  Pabcp=[10e3 9e3 11e3]  QLabcp=[100 90 110]  QCabcp=[100 90 110]  Measurements=None  LoadType=constant Z
  Load 894 : spsThreePhaseSeriesRLCLoadLib/Three-Phase Series RLC Load  LConnTagsString=A|B|C  Configuration=Delta  NominalVoltage=10000  Vabc=[1e3 1e3 1e3]  Vabcp=[1e3 1e3 1e3]  NominalFrequency=50  UnbalancedPower=off  ActivePower=3246.7774  InductivePower=1258.5349  CapacitivePower=0  Pabc=[10e3 9e3 11e3]  QLabc=[100 90 110]  QCabc=[100 90 110]  Pabcp=[10e3 9e3 11e3]  QLabcp=[100 90 110]  QCabcp=[100 90 110]  Measurements=None  LoadType=constant Z
  Load 895 : spsThreePhaseSeriesRLCLoadLib/Three-Phase Series RLC Load  LConnTagsString=A|B|C  Configuration=Delta  NominalVoltage=10000  Vabc=[1e3 1e3 1e3]  Vabcp=[1e3 1e3 1e3]  NominalFrequency=50  UnbalancedPower=off  ActivePower=1257.9477  InductivePower=324.0486  CapacitivePower=0  Pabc=[10e3 9e3 11e3]  QLabc=[100 90 110]  QCabc=[100 90 110]  Pabcp=[10e3 9e3 11e3]  QLabcp=[100 90 110]  QCabcp=[100 90 110]  Measurements=None  LoadType=constant Z
  R1 : spsThreePhaseVIMeasurementLib/Three-Phase V-I Measurement  VoltageMeasurement=phase-to-ground  SetLabelV=off  LabelV=Vabc  Vpu=off  VpuLL=off  CurrentMeasurement=yes  SetLabelI=off  LabelI=Iabc  Ipu=off  Pbase=100e6  Vbase=500e3  OutputType=Complex  PhasorSimulation=on  PSBequivalent=0
  R4 : spsThreePhaseVIMeasurementLib/Three-Phase V-I Measurement  VoltageMeasurement=phase-to-ground  SetLabelV=off  LabelV=Vabc  Vpu=off  VpuLL=off  CurrentMeasurement=yes  SetLabelI=off  LabelI=Iabc  Ipu=off  Pbase=100e6  Vbase=500e3  OutputType=Complex  PhasorSimulation=on  PSBequivalent=0
  R6 : spsThreePhaseVIMeasurementLib/Three-Phase V-I Measurement  VoltageMeasurement=phase-to-ground  SetLabelV=off  LabelV=Vabc  Vpu=off  VpuLL=off  CurrentMeasurement=yes  SetLabelI=off  LabelI=Iabc  Ipu=off  Pbase=100e6  Vbase=500e3  OutputType=Complex  PhasorSimulation=on  PSBequivalent=0
  Scope R1 : Scope  NumInputPorts=2
  Scope R4 : Scope  NumInputPorts=2
  Scope R6 : Scope  NumInputPorts=2
  Source PC1_TT2 : spsThreePhaseSourceLib/Three-Phase Source  InternalConnection=Yn  VoltagePhases=off  Voltage=10000  PhaseAngle=0  Voltage_phases=[25e3 25e3 25e3]/sqrt(3)  PhaseAngles_phases=[0 -120 +120]  Frequency=50  NonIdealSource=on  SpecifyImpedance=off  Resistance=0.14  Inductance=0.0031831  ShortCircuitLevel=100e6  BaseVoltage=25e3  XRratio=7  BusType=swing  Pref=10e3  Qref=0  Prefabc=[10e3, 10e3, 10e3]  Qrefabc=[0, 0, 0]  Qmin=-inf  Qmax=inf
  Source Zn : spsSeriesRLCBranchLib/Series RLC Branch  LConnTagsString=__new0  RConnTagsString=__new0  BranchType=RL  Resistance=0.001  Inductance=3.1831e-06  SetiL0=off  InitialCurrent=0  Capacitance=0  Setx0=off  InitialVoltage=0  Measurements=None
  powergui : spspowerguiLib/powergui  Priority=1  SimulationMode=Phasor  SampleTime=50e-6  frequency=50  Iterations=50  frequencyindice=50  Pbase=100e6  ErrMax=1e-4  UnitsV=kV  UnitsW=MW  buscounter=0  FunctionMessages=off  echomessages=off  EnableUseOfTLC=off  CurrentSourceSwitches=off  DisableSnubberDevices=off  DisableRonSwitches=off  DisableVfSwitches=off  DisplayEquations=off  AutomaticDiscreteSolvers=off  SolverType=Tustin/Backward Euler (TBE)  Interpol=off  ExternalGateDelay=off  methode=off  Ts=10  x0status=blocks  SPID=off  SwTol=0  HookPort=off  NonlinearTolerance=1e-4  nMaxIteration=100  ContinueOnMaxIteration=off  RestoreLinks=warning  ResistiveCurrentMeasurement=off  Frange=[0:2:500]  Ylog=off  Xlog=on  ShowGrid=off  save=off  variable=ZData  structure=0  ZoomFFT=off  StartTime=0.0  cycles=1  DisplayStyle=1  fundamental=60  FreqAxis=off  MaxFrequency=1000  frequencyindicesteady=1  RmsSteady=1  display=off
  wires:
  R6/1 -> Scope R6/1
  R6/2 -> Scope R6/2
  R4/1 -> Scope R4/1
  R4/2 -> Scope R4/2
  R1/1 -> Scope R1/1
  R1/2 -> Scope R1/2
  connections:
  Ground/LConn1 -- Source Zn/LConn1
  Source Zn/RConn1 -- Source PC1_TT2/LConn1
  Line 6/LConn1 -- Line 4/RConn1 -- Line 5/LConn1
  Line 6/LConn2 -- Line 4/RConn2 -- Line 5/LConn2
  Line 6/LConn3 -- Line 4/RConn3 -- Line 5/LConn3
  Line 21/RConn1 -- Line 22/LConn1
  Line 21/RConn2 -- Line 22/LConn2
  Line 21/RConn3 -- Line 22/LConn3
  Line 25/LConn1 -- Line 24/RConn1
  Line 25/LConn2 -- Line 24/RConn2
  Line 25/LConn3 -- Line 24/RConn3
  Line 28/RConn1 -- Load 8590/LConn1
  Line 28/RConn2 -- Load 8590/LConn2
  Line 28/RConn3 -- Load 8590/LConn3
  Line 11/RConn1 -- Load 174/LConn1
  Line 11/RConn2 -- Load 174/LConn2
  Line 11/RConn3 -- Load 174/LConn3
  Load 8478/LConn1 -- Line 37/RConn1
  Load 8478/LConn2 -- Line 37/RConn2
  Load 8478/LConn3 -- Line 37/RConn3
  Line/RConn1 -- R1/LConn1
  Line/RConn2 -- R1/LConn2
  Line/RConn3 -- R1/LConn3
  Line 14/LConn1 -- Line 13/LConn1 -- Line 12/RConn1
  Line 14/LConn2 -- Line 13/LConn2 -- Line 12/RConn2
  Line 14/LConn3 -- Line 13/LConn3 -- Line 12/RConn3
  Line 43/RConn1 -- Load 8693/LConn1
  Line 43/RConn2 -- Load 8693/LConn2
  Line 43/RConn3 -- Load 8693/LConn3
  Load 8202/LConn1 -- Line 26/LConn1 -- Line 25/RConn1
  Load 8202/LConn2 -- Line 26/LConn2 -- Line 25/RConn2
  Load 8202/LConn3 -- Line 26/LConn3 -- Line 25/RConn3
  Line im1/LConn1 -- R4/RConn1
  Line im1/LConn2 -- R4/RConn2
  Line im1/LConn3 -- R4/RConn3
  Line 21/LConn1 -- Line 20/RConn1
  Line 21/LConn2 -- Line 20/RConn2
  Line 21/LConn3 -- Line 20/RConn3
  Line 43/LConn1 -- Line 42/LConn1 -- Line 41/RConn1
  Line 43/LConn2 -- Line 42/LConn2 -- Line 41/RConn2
  Line 43/LConn3 -- Line 42/LConn3 -- Line 41/RConn3
  Line 35/LConn1 -- Load 8131/LConn1 -- Line im1/RConn1
  Line 35/LConn2 -- Load 8131/LConn2 -- Line im1/RConn2
  Line 35/LConn3 -- Load 8131/LConn3 -- Line im1/RConn3
  Line 38/LConn1 -- Line 37/LConn1 -- Line 36/RConn1
  Line 38/LConn2 -- Line 37/LConn2 -- Line 36/RConn2
  Line 38/LConn3 -- Line 37/LConn3 -- Line 36/RConn3
  Line 7/RConn1 -- Load 535/LConn1
  Line 7/RConn2 -- Load 535/LConn2
  Line 7/RConn3 -- Load 535/LConn3
  Line 24/LConn1 -- Line 23/RConn1
  Line 24/LConn2 -- Line 23/RConn2
  Line 24/LConn3 -- Line 23/RConn3
  Line 18/RConn1 -- Line 19/LConn1
  Line 18/RConn2 -- Line 19/LConn2
  Line 18/RConn3 -- Line 19/LConn3
  Source PC1_TT2/RConn1 -- Line/LConn1
  Source PC1_TT2/RConn2 -- Line/LConn2
  Source PC1_TT2/RConn3 -- Line/LConn3
  Line 7/LConn1 -- Line 6/RConn1
  Line 7/LConn2 -- Line 6/RConn2
  Line 7/LConn3 -- Line 6/RConn3
  Line 5/RConn1 -- Load 534/LConn1
  Line 5/RConn2 -- Load 534/LConn2
  Line 5/RConn3 -- Load 534/LConn3
  Line 10/LConn1 -- Line 15/LConn1 -- Line 9/LConn1 -- Line 8/RConn1
  Line 10/LConn2 -- Line 15/LConn2 -- Line 9/LConn2 -- Line 8/RConn2
  Line 10/LConn3 -- Line 15/LConn3 -- Line 9/LConn3 -- Line 8/RConn3
  Line 30/RConn1 -- Load 171/LConn1
  Line 30/RConn2 -- Load 171/LConn2
  Line 30/RConn3 -- Load 171/LConn3
  Line 34/LConn1 -- Line 18/LConn1 -- Line 17/RConn1
  Line 34/LConn2 -- Line 18/LConn2 -- Line 17/RConn2
  Line 34/LConn3 -- Line 18/LConn3 -- Line 17/RConn3
  Load 178/LConn1 -- Line 3/LConn1 -- Line 2/RConn1
  Load 178/LConn2 -- Line 3/LConn2 -- Line 2/RConn2
  Load 178/LConn3 -- Line 3/LConn3 -- Line 2/RConn3
  Line 14/RConn1 -- Load 895/LConn1
  Line 14/RConn2 -- Load 895/LConn2
  Line 14/RConn3 -- Load 895/LConn3
  Load 1873/LConn1 -- Line 9/RConn1
  Load 1873/LConn2 -- Line 9/RConn2
  Load 1873/LConn3 -- Line 9/RConn3
  Line 32/RConn1 -- Load 8468/LConn1
  Line 32/RConn2 -- Load 8468/LConn2
  Line 32/RConn3 -- Load 8468/LConn3
  Line 29/LConn1 -- Line 28/LConn1 -- Line 27/RConn1
  Line 29/LConn2 -- Line 28/LConn2 -- Line 27/RConn2
  Line 29/LConn3 -- Line 28/LConn3 -- Line 27/RConn3
  Line 41/LConn1 -- Line 40/LConn1 -- Line 39/RConn1
  Line 41/LConn2 -- Line 40/LConn2 -- Line 39/RConn2
  Line 41/LConn3 -- Line 40/LConn3 -- Line 39/RConn3
  Line im2/LConn1 -- Line 39/LConn1 -- Line 38/RConn1
  Line im2/LConn2 -- Line 39/LConn2 -- Line 38/RConn2
  Line im2/LConn3 -- Line 39/LConn3 -- Line 38/RConn3
  Line 40/RConn1 -- Load 8130/LConn1
  Line 40/RConn2 -- Load 8130/LConn2
  Line 40/RConn3 -- Load 8130/LConn3
  Line 33/LConn1 -- Line 32/LConn1 -- Line 31/RConn1
  Line 33/LConn2 -- Line 32/LConn2 -- Line 31/RConn2
  Line 33/LConn3 -- Line 32/LConn3 -- Line 31/RConn3
  Line 33/RConn1 -- R6/LConn1
  Line 33/RConn2 -- R6/LConn2
  Line 33/RConn3 -- R6/LConn3
  Line 8/LConn1 -- Line 4/LConn1 -- Line 3/RConn1
  Line 8/LConn2 -- Line 4/LConn2 -- Line 3/RConn2
  Line 8/LConn3 -- Line 4/LConn3 -- Line 3/RConn3
  Line 36/LConn1 -- Line 35/RConn1
  Line 36/LConn2 -- Line 35/RConn2
  Line 36/LConn3 -- Line 35/RConn3
  Line 13/RConn1 -- Load 894/LConn1
  Line 13/RConn2 -- Load 894/LConn2
  Line 13/RConn3 -- Load 894/LConn3
  Load 8193/LConn1 -- Line 31/LConn1 -- Line 30/LConn1 -- Line 29/RConn1
  Load 8193/LConn2 -- Line 31/LConn2 -- Line 30/LConn2 -- Line 29/RConn2
  Load 8193/LConn3 -- Line 31/LConn3 -- Line 30/LConn3 -- Line 29/RConn3
  Line 17/LConn1 -- Line 16/LConn1 -- Line 15/RConn1
  Line 17/LConn2 -- Line 16/LConn2 -- Line 15/RConn2
  Line 17/LConn3 -- Line 16/LConn3 -- Line 15/RConn3
  Line 2/LConn1 -- R1/RConn1
  Line 2/LConn2 -- R1/RConn2
  Line 2/LConn3 -- R1/RConn3
  Line 26/RConn1 -- Line 27/LConn1
  Line 26/RConn2 -- Line 27/LConn2
  Line 26/RConn3 -- Line 27/LConn3
  Load 8201/LConn1 -- Line 42/RConn1
  Load 8201/LConn2 -- Line 42/RConn2
  Load 8201/LConn3 -- Line 42/RConn3
  Line 23/LConn1 -- Load 8624/LConn1 -- Line 22/RConn1
  Line 23/LConn2 -- Load 8624/LConn2 -- Line 22/RConn2
  Line 23/LConn3 -- Load 8624/LConn3 -- Line 22/RConn3
  Line 11/LConn1 -- Line 12/LConn1 -- Line 10/RConn1
  Line 11/LConn2 -- Line 12/LConn2 -- Line 10/RConn2
  Line 11/LConn3 -- Line 12/LConn3 -- Line 10/RConn3
  Line 34/RConn1 -- R4/LConn1
  Line 34/RConn2 -- R4/LConn2
  Line 34/RConn3 -- R4/LConn3
  Load 8042/LConn1 -- Line 16/RConn1
  Load 8042/LConn2 -- Line 16/RConn2
  Load 8042/LConn3 -- Line 16/RConn3
  Load 8429/LConn1 -- Line 20/LConn1 -- Line 19/RConn1
  Load 8429/LConn2 -- Line 20/LConn2 -- Line 19/RConn2
  Load 8429/LConn3 -- Line 20/LConn3 -- Line 19/RConn3
